simulink library "ammclib_bam_S32K3xx"  (R2016a)
(part 16 of 50)

      |   f32PropGainQ=round(kpf*2^(-s16PropGainShiftQ)*2^31);
      |   if f32PropGainQ>2^31-1
      |     f32PropGainQ=2^31-1;
      |     warning(['Parameter f32PropGainQ of ' gcb ' exceeds the fixed-point range.']);
      |   end
      |   if f32PropGainQ<-2^31
      |     f32PropGainQ=-2^31;
      |     warning(['Parameter f32PropGainQ of ' gcb ' exceeds the fixed-point range.']);
      |   end
      |   kif=igain*SampleTime*0.5*wmax/iscale;
      |   s16IntegGainShiftQ=ceil(log2(abs(kif)));
      |   if s16IntegGainShiftQ<-31
      |     s16IntegGainShiftQ=-31;
      |   end
      |   if s16IntegGainShiftQ>31
      |     s16IntegGainShiftQ=31;
      |     warning(['Parameter s16IntegGainShiftQ of ' gcb ' exceeds the fixed-point range.']);
      |   end
      |   f32IntegGainQ=round(kif*2^(-s16IntegGainShiftQ)*2^31);
      |   if f32IntegGainQ>2^31-1
      |     f32IntegGainQ=2^31-1;
      |     warning(['Parameter f32IntegGainQ of ' gcb ' exceeds the fixed-point range.']);
      |   end
      |   if f32IntegGainQ<-2^31
      |     f32IntegGainQ=-2^31;
      |     warning(['Parameter f32IntegGainQ of ' gcb ' exceeds the fixed-point range.']);
      |   end
      |   f32LowerLimitQ=-2147483648;
      |   f32UpperLimitQ=2147483647;
      |   fwkpf=0.9*pgain*wmax/iscale;
      |   s16PropGainShiftFW=ceil(log2(abs(fwkpf)));
      |   if s16PropGainShiftFW<-31
      |     s16PropGainShiftFW=-31;
      |   end
      |   if s16PropGainShiftFW>31
      |     s16PropGainShiftFW=31;
      |     warning(['Parameter s16PropGainShiftFW of ' gcb ' exceeds the fixed-point range.']);
      |   end
      |   f32PropGainFW=round(fwkpf*2^(-s16PropGainShiftFW)*2^31);
      |   if f32PropGainFW>2^31-1
      |     f32PropGainFW=2^31-1;
      |     warning(['Parameter f32PropGainFW of ' gcb ' exceeds the fixed-point range.']);
      |   end
      |   if f32PropGainFW<-2^31
      |     f32PropGainFW=-2^31;
      |     warning(['Parameter f32PropGainFW of ' gcb ' exceeds the fixed-point range.']);
      |   end
      |   s16IntegGainShiftFW=s16IntegGainShiftQ;
      |   f32IntegGainFW=f32IntegGainQ;
      |   if (Idmax<0)
      |     iratio=abs(Idmax)/iscale;
      |     if (abs(iratio) > 1)
      |       iratio = 0;
      |     end
      |     lowlim=0.3183098861837907*acos(iratio)-0.5;
      |   else
      |     lowlim=0.0;
      |   end
      |   f32LowerLimitFW=round(lowlim*2^31);
      |   if f32LowerLimitFW>2^31-1
      |     f32LowerLimitFW=2^31-1;
      |     warning(['Parameter f32LowerLimitFW of ' gcb ' exceeds the fixed-point range.']);
      |   end
      |   if f32LowerLimitFW<-2^31
      |     f32LowerLimitFW=-2^31;
      |     warning(['Parameter f32LowerLimitFW of ' gcb ' exceeds the fixed-point range.']);
      |   end
      |   f32UpperLimitFW=0;
      |   u16NSamplesW=round(log2(1.0/abs(lambdaW)));
      |   if u16NSamplesW>31
      |     u16NSamplesW=31;
      |   end
      |   if u16NSamplesW<0
      |     u16NSamplesW=0;
      |   end
      |   u16NSamplesFW=round(log2(1.0/abs(lambdaFW)));
      |   if u16NSamplesFW>31
      |     u16NSamplesFW=31;
      |   end
      |   if u16NSamplesFW<0
      |     u16NSamplesFW=0;
      |   end
      |   rampsc=polepairs*abs(ramprpm)*0.1047197551196598/wmax;
      |   f32RampUp=round(rampsc*2^31);
      |   if f32RampUp>2^31-1
      |     f32RampUp=2^31-1;
      |     warning(['Parameter f32RampUp of ' gcb ' exceeds the fixed-point range.']);
      |   end
      |   if f32RampUp<-2^31
      |     f32RampUp=-2^31;
      |     warning(['Parameter f32RampUp of ' gcb ' exceeds the fixed-point range.']);
      |   end
      |   f32RampDown=round(rampsc*2^31);
      |   if f32RampDown>2^31-1
      |     f32RampDown=2^31-1;
      |     warning(['Parameter f32RampDown of ' gcb ' exceeds the fixed-point range.']);
      |   end
      |   if f32RampDown<-2^31
      |     f32RampDown=-2^31;
      |     warning(['Parameter f32RampDown of ' gcb ' exceeds the fixed-point range.']);
      |   end
      |   if isnan(u16NSamplesW)
      |     if ~strcmp(u16NSamplesW_bkup,'0')
      |       set_param(gcb,'u16NSamplesW','0');
      |     end
      |   else
      |     tmps=num2str(u16NSamplesW);
      |     if ~strcmp(u16NSamplesW_bkup,tmps)
      |       set_param(gcb,'u16NSamplesW',tmps);
      |     end
      |   end
      |   if isnan(u16NSamplesFW)
      |     if ~strcmp(u16NSamplesFW_bkup,'0')
      |       set_param(gcb,'u16NSamplesFW','0');
      |     end
      |   else
      |     tmps=num2str(u16NSamplesFW);
      |     if ~strcmp(u16NSamplesFW_bkup,tmps)
      |       set_param(gcb,'u16NSamplesFW',tmps);
      |     end
      |   end
      |   if isnan(f32PropGainQ)
      |     if ~strcmp(f32PropGainQ_bkup,'0')
      |       set_param(gcb,'f32PropGainQ','0');
      |     end
      |   else
      |     tmps=num2str(f32PropGainQ);
      |     if ~strcmp(f32PropGainQ_bkup,tmps)
      |       set_param(gcb,'f32PropGainQ',tmps);
      |     end
      |   end
      |   if isnan(f32IntegGainQ)
      |     if ~strcmp(f32IntegGainQ_bkup,'0')
      |       set_param(gcb,'f32IntegGainQ','0');
      |     end
      |   else
      |     tmps=num2str(f32IntegGainQ);
      |     if ~strcmp(f32IntegGainQ_bkup,tmps)
      |       set_param(gcb,'f32IntegGainQ',tmps);
      |     end
      |   end
      |   if isnan(s16PropGainShiftQ)
      |     if ~strcmp(s16PropGainShiftQ_bkup,'0')
      |       set_param(gcb,'s16PropGainShiftQ','0');
      |     end
      |   else
      |     tmps=num2str(s16PropGainShiftQ);
      |     if ~strcmp(s16PropGainShiftQ_bkup,tmps)
      |       set_param(gcb,'s16PropGainShiftQ',tmps);
      |     end
      |   end
      |   if isnan(s16IntegGainShiftQ)
      |     if ~strcmp(s16IntegGainShiftQ_bkup,'0')
      |       set_param(gcb,'s16IntegGainShiftQ','0');
      |     end
      |   else
      |     tmps=num2str(s16IntegGainShiftQ);
      |     if ~strcmp(s16IntegGainShiftQ_bkup,tmps)
      |       set_param(gcb,'s16IntegGainShiftQ',tmps);
      |     end
      |   end
      |   if isnan(f32LowerLimitQ)
      |     if ~strcmp(f32LowerLimitQ_bkup,'0')
      |       set_param(gcb,'f32LowerLimitQ','0');
      |     end
      |   else
      |     tmps=num2str(f32LowerLimitQ);
      |     if ~strcmp(f32LowerLimitQ_bkup,tmps)
      |       set_param(gcb,'f32LowerLimitQ',tmps);
      |     end
      |   end
      |   if isnan(f32UpperLimitQ)
      |     if ~strcmp(f32UpperLimitQ_bkup,'0')
      |       set_param(gcb,'f32UpperLimitQ','0');
      |     end
      |   else
      |     tmps=num2str(f32UpperLimitQ);
      |     if ~strcmp(f32UpperLimitQ_bkup,tmps)
      |       set_param(gcb,'f32UpperLimitQ',tmps);
      |     end
      |   end
      |   if isnan(f32PropGainFW)
      |     if ~strcmp(f32PropGainFW_bkup,'0')
      |       set_param(gcb,'f32PropGainFW','0');
      |     end
      |   else
      |     tmps=num2str(f32PropGainFW);
      |     if ~strcmp(f32PropGainFW_bkup,tmps)
      |       set_param(gcb,'f32PropGainFW',tmps);
      |     end
      |   end
      |   if isnan(f32IntegGainFW)
      |     if ~strcmp(f32IntegGainFW_bkup,'0')
      |       set_param(gcb,'f32IntegGainFW','0');
      |     end
      |   else
      |     tmps=num2str(f32IntegGainFW);
      |     if ~strcmp(f32IntegGainFW_bkup,tmps)
      |       set_param(gcb,'f32IntegGainFW',tmps);
      |     end
      |   end
      |   if isnan(s16PropGainShiftFW)
      |     if ~strcmp(s16PropGainShiftFW_bkup,'0')
      |       set_param(gcb,'s16PropGainShiftFW','0');
      |     end
      |   else
      |     tmps=num2str(s16PropGainShiftFW);
      |     if ~strcmp(s16PropGainShiftFW_bkup,tmps)
      |       set_param(gcb,'s16PropGainShiftFW',tmps);
      |     end
      |   end
      |   if isnan(s16IntegGainShiftFW)
      |     if ~strcmp(s16IntegGainShiftFW_bkup,'0')
      |       set_param(gcb,'s16IntegGainShiftFW','0');
      |     end
      |   else
      |     tmps=num2str(s16IntegGainShiftFW);
      |     if ~strcmp(s16IntegGainShiftFW_bkup,tmps)
      |       set_param(gcb,'s16IntegGainShiftFW',tmps);
      |     end
      |   end
      |   if isnan(f32LowerLimitFW)
      |     if ~strcmp(f32LowerLimitFW_bkup,'0')
      |       set_param(gcb,'f32LowerLimitFW','0');
      |     end
      |   else
      |     tmps=num2str(f32LowerLimitFW);
      |     if ~strcmp(f32LowerLimitFW_bkup,tmps)
      |       set_param(gcb,'f32LowerLimitFW',tmps);
      |     end
      |   end
      |   if isnan(f32UpperLimitFW)
      |     if ~strcmp(f32UpperLimitFW_bkup,'0')
      |       set_param(gcb,'f32UpperLimitFW','0');
      |     end
      |   else
      |     tmps=num2str(f32UpperLimitFW);
      |     if ~strcmp(f32UpperLimitFW_bkup,tmps)
      |       set_param(gcb,'f32UpperLimitFW',tmps);
      |     end
      |   end
      |   if isnan(f32RampUp)
      |     if ~strcmp(f32RampUp_bkup,'0')
      |       set_param(gcb,'f32RampUp','0');
      |     end
      |   else
      |     tmps=num2str(f32RampUp);
      |     if ~strcmp(f32RampUp_bkup,tmps)
      |       set_param(gcb,'f32RampUp',tmps);
      |     end
      |   end
      |   if isnan(f32RampDown)
      |     if ~strcmp(f32RampDown_bkup,'0')
      |       set_param(gcb,'f32RampDown','0');
      |     end
      |   else
      |     tmps=num2str(f32RampDown);
      |     if ~strcmp(f32RampDown_bkup,tmps)
      |       set_param(gcb,'f32RampDown',tmps);
      |     end
      |   end
      | end
      mask Callback J:
      | autoCalcEn=get_param(gcb,'autoCalcEn');
      | if strcmp(autoCalcEn,'on')
      |   SampleTime=Simulink.data.evalinGlobal(bdroot,get_param(gcb,'SampleTime'));
      |   if (SampleTime==-1)
      |     SampleTime=str2double(get_param(gcb,'SampleTime_1'));
      |   end
      |   u16NSamplesW_bkup=get_param(gcb,'u16NSamplesW');
      |   u16NSamplesFW_bkup=get_param(gcb,'u16NSamplesFW');
      |   f32PropGainQ_bkup=get_param(gcb,'f32PropGainQ');
      |   f32IntegGainQ_bkup=get_param(gcb,'f32IntegGainQ');
      |   s16PropGainShiftQ_bkup=get_param(gcb,'s16PropGainShiftQ');
      |   s16IntegGainShiftQ_bkup=get_param(gcb,'s16IntegGainShiftQ');
      |   f32LowerLimitQ_bkup=get_param(gcb,'f32LowerLimitQ');
      |   f32UpperLimitQ_bkup=get_param(gcb,'f32UpperLimitQ');
      |   f32PropGainFW_bkup=get_param(gcb,'f32PropGainFW');
      |   f32IntegGainFW_bkup=get_param(gcb,'f32IntegGainFW');
      |   s16PropGainShiftFW_bkup=get_param(gcb,'s16PropGainShiftFW');
      |   s16IntegGainShiftFW_bkup=get_param(gcb,'s16IntegGainShiftFW');
      |   f32LowerLimitFW_bkup=get_param(gcb,'f32LowerLimitFW');
      |   f32UpperLimitFW_bkup=get_param(gcb,'f32UpperLimitFW');
      |   f32RampUp_bkup=get_param(gcb,'f32RampUp');
      |   f32RampDown_bkup=get_param(gcb,'f32RampDown');
      |   wf0=Simulink.data.evalinGlobal(bdroot,get_param(gcb,'wf0'));
      |   wksi=Simulink.data.evalinGlobal(bdroot,get_param(gcb,'wksi'));
      |   J=Simulink.data.evalinGlobal(bdroot,get_param(gcb,'J'));
      |   Kt=Simulink.data.evalinGlobal(bdroot,get_param(gcb,'Kt'));
      |   lambdaW=Simulink.data.evalinGlobal(bdroot,get_param(gcb,'lambdaW'));
      |   lambdaFW=Simulink.data.evalinGlobal(bdroot,get_param(gcb,'lambdaFW'));
      |   Idmax=Simulink.data.evalinGlobal(bdroot,get_param(gcb,'Idmax'));
      |   ramprpm=Simulink.data.evalinGlobal(bdroot,get_param(gcb,'ramprpm'));
      |   mechspeed=Simulink.data.evalinGlobal(bdroot,get_param(gcb,'mechspeed'));
      |   polepairs=Simulink.data.evalinGlobal(bdroot,get_param(gcb,'polepairs'));
      |   uscale=Simulink.data.evalinGlobal(bdroot,get_param(gcb,'uscale'));
      |   iscale=Simulink.data.evalinGlobal(bdroot,get_param(gcb,'iscale'));
      |   if (wf0<=0)
      |     warning('Natural frequency f0 must be positive.');
      |   end
      |   if (wksi<=0)
      |     warning('Current loop attenuation must be positive.');
      |   end
      |   if (wksi>1)
      |     warning('Current loop attenuation must not exceed 1.');
      |   end
      |   if (J<=0)
      |     warning('Moment of inertia J must be positive.');
      |   end
      |   if (Kt<=0)
      |     warning('Torque constant Kt must be positive.');
      |   end
      |   if (lambdaW<0)
      |     warning('MA filter smoothing factor must be in the range 0..1.');
      |   end
      |   if (lambdaW>1)
      |     warning('MA filter smoothing factor must be in the range 0..1.');
      |   end
      |   if (lambdaFW<0)
      |     warning('MA filter smoothing factor must be in the range 0..1.');
      |   end
      |   if (lambdaFW>1)
      |     warning('MA filter smoothing factor must be in the range 0..1.');
      |   end
      |   if (mechspeed<=0)
      |     warning('Max. speed must be positive.');
      |   end
      |   if (polepairs<1)
      |     warning('Number of pole pairs must be a natural number (1, 2, 3, ...).');
      |   end
      |   if (round(polepairs)~=polepairs)
      |     warning('Number of pole pairs must be a natural number (1, 2, 3, ...).');
      |   end
      |   if (uscale<=0)
      |     warning('U_max must be positive.');
      |   end
      |   if (iscale<=0)
      |     warning('I_max must be positive.');
      |   end
      |   w0=6.283185307179586*wf0;
      |   pgain=2.0*wksi*w0*J/Kt;
      |   igain=w0*w0*J/Kt;
      |   wmax=polepairs*mechspeed*0.1047197551196598;
      |   kpf=pgain*wmax/iscale;
      |   s16PropGainShiftQ=ceil(log2(abs(kpf)));
      |   if s16PropGainShiftQ<-31
      |     s16PropGainShiftQ=-31;
      |   end
      |   if s16PropGainShiftQ>31
      |     s16PropGainShiftQ=31;
      |     warning(['Parameter s16PropGainShiftQ of ' gcb ' exceeds the fixed-point range.']);
      |   end
      |   f32PropGainQ=round(kpf*2^(-s16PropGainShiftQ)*2^31);
      |   if f32PropGainQ>2^31-1
      |     f32PropGainQ=2^31-1;
      |     warning(['Parameter f32PropGainQ of ' gcb ' exceeds the fixed-point range.']);
      |   end
      |   if f32PropGainQ<-2^31
      |     f32PropGainQ=-2^31;
      |     warning(['Parameter f32PropGainQ of ' gcb ' exceeds the fixed-point range.']);
      |   end
      |   kif=igain*SampleTime*0.5*wmax/iscale;
      |   s16IntegGainShiftQ=ceil(log2(abs(kif)));
      |   if s16IntegGainShiftQ<-31
      |     s16IntegGainShiftQ=-31;
      |   end
      |   if s16IntegGainShiftQ>31
      |     s16IntegGainShiftQ=31;
      |     warning(['Parameter s16IntegGainShiftQ of ' gcb ' exceeds the fixed-point range.']);
      |   end
      |   f32IntegGainQ=round(kif*2^(-s16IntegGainShiftQ)*2^31);
      |   if f32IntegGainQ>2^31-1
      |     f32IntegGainQ=2^31-1;
      |     warning(['Parameter f32IntegGainQ of ' gcb ' exceeds the fixed-point range.']);
      |   end
      |   if f32IntegGainQ<-2^31
      |     f32IntegGainQ=-2^31;
      |     warning(['Parameter f32IntegGainQ of ' gcb ' exceeds the fixed-point range.']);
      |   end
      |   f32LowerLimitQ=-2147483648;
      |   f32UpperLimitQ=2147483647;
      |   fwkpf=0.9*pgain*wmax/iscale;
      |   s16PropGainShiftFW=ceil(log2(abs(fwkpf)));
      |   if s16PropGainShiftFW<-31
      |     s16PropGainShiftFW=-31;
      |   end
      |   if s16PropGainShiftFW>31
      |     s16PropGainShiftFW=31;
      |     warning(['Parameter s16PropGainShiftFW of ' gcb ' exceeds the fixed-point range.']);
      |   end
      |   f32PropGainFW=round(fwkpf*2^(-s16PropGainShiftFW)*2^31);
      |   if f32PropGainFW>2^31-1
      |     f32PropGainFW=2^31-1;
      |     warning(['Parameter f32PropGainFW of ' gcb ' exceeds the fixed-point range.']);
      |   end
      |   if f32PropGainFW<-2^31
      |     f32PropGainFW=-2^31;
      |     warning(['Parameter f32PropGainFW of ' gcb ' exceeds the fixed-point range.']);
      |   end
      |   s16IntegGainShiftFW=s16IntegGainShiftQ;
      |   f32IntegGainFW=f32IntegGainQ;
      |   if (Idmax<0)
      |     iratio=abs(Idmax)/iscale;
      |     if (abs(iratio) > 1)
      |       iratio = 0;
      |     end
      |     lowlim=0.3183098861837907*acos(iratio)-0.5;
      |   else
      |     lowlim=0.0;
      |   end
      |   f32LowerLimitFW=round(lowlim*2^31);
      |   if f32LowerLimitFW>2^31-1
      |     f32LowerLimitFW=2^31-1;
      |     warning(['Parameter f32LowerLimitFW of ' gcb ' exceeds the fixed-point range.']);
      |   end
      |   if f32LowerLimitFW<-2^31
      |     f32LowerLimitFW=-2^31;
      |     warning(['Parameter f32LowerLimitFW of ' gcb ' exceeds the fixed-point range.']);
      |   end
      |   f32UpperLimitFW=0;
      |   u16NSamplesW=round(log2(1.0/abs(lambdaW)));
      |   if u16NSamplesW>31
      |     u16NSamplesW=31;
      |   end
      |   if u16NSamplesW<0
      |     u16NSamplesW=0;
      |   end
      |   u16NSamplesFW=round(log2(1.0/abs(lambdaFW)));
      |   if u16NSamplesFW>31
      |     u16NSamplesFW=31;
      |   end
      |   if u16NSamplesFW<0
      |     u16NSamplesFW=0;
      |   end
      |   rampsc=polepairs*abs(ramprpm)*0.1047197551196598/wmax;
      |   f32RampUp=round(rampsc*2^31);
      |   if f32RampUp>2^31-1
      |     f32RampUp=2^31-1;
      |     warning(['Parameter f32RampUp of ' gcb ' exceeds the fixed-point range.']);
      |   end
      |   if f32RampUp<-2^31
      |     f32RampUp=-2^31;
      |     warning(['Parameter f32RampUp of ' gcb ' exceeds the fixed-point range.']);
      |   end
      |   f32RampDown=round(rampsc*2^31);
      |   if f32RampDown>2^31-1
      |     f32RampDown=2^31-1;
      |     warning(['Parameter f32RampDown of ' gcb ' exceeds the fixed-point range.']);
      |   end
      |   if f32RampDown<-2^31
      |     f32RampDown=-2^31;
      |     warning(['Parameter f32RampDown of ' gcb ' exceeds the fixed-point range.']);
      |   end
      |   if isnan(u16NSamplesW)
      |     if ~strcmp(u16NSamplesW_bkup,'0')
      |       set_param(gcb,'u16NSamplesW','0');
      |     end
      |   else
      |     tmps=num2str(u16NSamplesW);
      |     if ~strcmp(u16NSamplesW_bkup,tmps)
      |       set_param(gcb,'u16NSamplesW',tmps);
      |     end
      |   end
      |   if isnan(u16NSamplesFW)
      |     if ~strcmp(u16NSamplesFW_bkup,'0')
      |       set_param(gcb,'u16NSamplesFW','0');
      |     end
      |   else
      |     tmps=num2str(u16NSamplesFW);
      |     if ~strcmp(u16NSamplesFW_bkup,tmps)
      |       set_param(gcb,'u16NSamplesFW',tmps);
      |     end
      |   end
      |   if isnan(f32PropGainQ)
      |     if ~strcmp(f32PropGainQ_bkup,'0')
      |       set_param(gcb,'f32PropGainQ','0');
      |     end
      |   else
      |     tmps=num2str(f32PropGainQ);
      |     if ~strcmp(f32PropGainQ_bkup,tmps)
      |       set_param(gcb,'f32PropGainQ',tmps);
      |     end
      |   end
      |   if isnan(f32IntegGainQ)
      |     if ~strcmp(f32IntegGainQ_bkup,'0')
      |       set_param(gcb,'f32IntegGainQ','0');
      |     end
      |   else
      |     tmps=num2str(f32IntegGainQ);
      |     if ~strcmp(f32IntegGainQ_bkup,tmps)
      |       set_param(gcb,'f32IntegGainQ',tmps);
      |     end
      |   end
      |   if isnan(s16PropGainShiftQ)
      |     if ~strcmp(s16PropGainShiftQ_bkup,'0')
      |       set_param(gcb,'s16PropGainShiftQ','0');
      |     end
      |   else
      |     tmps=num2str(s16PropGainShiftQ);
      |     if ~strcmp(s16PropGainShiftQ_bkup,tmps)
      |       set_param(gcb,'s16PropGainShiftQ',tmps);
      |     end
      |   end
      |   if isnan(s16IntegGainShiftQ)
      |     if ~strcmp(s16IntegGainShiftQ_bkup,'0')
      |       set_param(gcb,'s16IntegGainShiftQ','0');
      |     end
      |   else
      |     tmps=num2str(s16IntegGainShiftQ);
      |     if ~strcmp(s16IntegGainShiftQ_bkup,tmps)
      |       set_param(gcb,'s16IntegGainShiftQ',tmps);
      |     end
      |   end
      |   if isnan(f32LowerLimitQ)
      |     if ~strcmp(f32LowerLimitQ_bkup,'0')
      |       set_param(gcb,'f32LowerLimitQ','0');
      |     end
      |   else
      |     tmps=num2str(f32LowerLimitQ);
      |     if ~strcmp(f32LowerLimitQ_bkup,tmps)
      |       set_param(gcb,'f32LowerLimitQ',tmps);
      |     end
      |   end
      |   if isnan(f32UpperLimitQ)
      |     if ~strcmp(f32UpperLimitQ_bkup,'0')
      |       set_param(gcb,'f32UpperLimitQ','0');
      |     end
      |   else
      |     tmps=num2str(f32UpperLimitQ);
      |     if ~strcmp(f32UpperLimitQ_bkup,tmps)
      |       set_param(gcb,'f32UpperLimitQ',tmps);
      |     end
      |   end
      |   if isnan(f32PropGainFW)
      |     if ~strcmp(f32PropGainFW_bkup,'0')
      |       set_param(gcb,'f32PropGainFW','0');
      |     end
      |   else
      |     tmps=num2str(f32PropGainFW);
      |     if ~strcmp(f32PropGainFW_bkup,tmps)
      |       set_param(gcb,'f32PropGainFW',tmps);
      |     end
      |   end
      |   if isnan(f32IntegGainFW)
      |     if ~strcmp(f32IntegGainFW_bkup,'0')
      |       set_param(gcb,'f32IntegGainFW','0');
      |     end
      |   else
      |     tmps=num2str(f32IntegGainFW);
      |     if ~strcmp(f32IntegGainFW_bkup,tmps)
      |       set_param(gcb,'f32IntegGainFW',tmps);
      |     end
      |   end
      |   if isnan(s16PropGainShiftFW)
      |     if ~strcmp(s16PropGainShiftFW_bkup,'0')
      |       set_param(gcb,'s16PropGainShiftFW','0');
      |     end
      |   else
      |     tmps=num2str(s16PropGainShiftFW);
      |     if ~strcmp(s16PropGainShiftFW_bkup,tmps)
      |       set_param(gcb,'s16PropGainShiftFW',tmps);
      |     end
      |   end
      |   if isnan(s16IntegGainShiftFW)
      |     if ~strcmp(s16IntegGainShiftFW_bkup,'0')
      |       set_param(gcb,'s16IntegGainShiftFW','0');
      |     end
      |   else
      |     tmps=num2str(s16IntegGainShiftFW);
      |     if ~strcmp(s16IntegGainShiftFW_bkup,tmps)
      |       set_param(gcb,'s16IntegGainShiftFW',tmps);
      |     end
      |   end
      |   if isnan(f32LowerLimitFW)
      |     if ~strcmp(f32LowerLimitFW_bkup,'0')
      |       set_param(gcb,'f32LowerLimitFW','0');
      |     end
      |   else
      |     tmps=num2str(f32LowerLimitFW);
      |     if ~strcmp(f32LowerLimitFW_bkup,tmps)
      |       set_param(gcb,'f32LowerLimitFW',tmps);
      |     end
      |   end
      |   if isnan(f32UpperLimitFW)
      |     if ~strcmp(f32UpperLimitFW_bkup,'0')
      |       set_param(gcb,'f32UpperLimitFW','0');
      |     end
      |   else
      |     tmps=num2str(f32UpperLimitFW);
      |     if ~strcmp(f32UpperLimitFW_bkup,tmps)
      |       set_param(gcb,'f32UpperLimitFW',tmps);
      |     end
      |   end
      |   if isnan(f32RampUp)
      |     if ~strcmp(f32RampUp_bkup,'0')
      |       set_param(gcb,'f32RampUp','0');
      |     end
      |   else
      |     tmps=num2str(f32RampUp);
      |     if ~strcmp(f32RampUp_bkup,tmps)
      |       set_param(gcb,'f32RampUp',tmps);
      |     end
      |   end
      |   if isnan(f32RampDown)
      |     if ~strcmp(f32RampDown_bkup,'0')
      |       set_param(gcb,'f32RampDown','0');
      |     end
      |   else
      |     tmps=num2str(f32RampDown);
      |     if ~strcmp(f32RampDown_bkup,tmps)
      |       set_param(gcb,'f32RampDown',tmps);
      |     end
      |   end
      | end
      mask Callback Kt:
      | autoCalcEn=get_param(gcb,'autoCalcEn');
      | if strcmp(autoCalcEn,'on')
      |   SampleTime=Simulink.data.evalinGlobal(bdroot,get_param(gcb,'SampleTime'));
      |   if (SampleTime==-1)
      |     SampleTime=str2double(get_param(gcb,'SampleTime_1'));
      |   end
      |   u16NSamplesW_bkup=get_param(gcb,'u16NSamplesW');
      |   u16NSamplesFW_bkup=get_param(gcb,'u16NSamplesFW');
      |   f32PropGainQ_bkup=get_param(gcb,'f32PropGainQ');
      |   f32IntegGainQ_bkup=get_param(gcb,'f32IntegGainQ');
      |   s16PropGainShiftQ_bkup=get_param(gcb,'s16PropGainShiftQ');
      |   s16IntegGainShiftQ_bkup=get_param(gcb,'s16IntegGainShiftQ');
      |   f32LowerLimitQ_bkup=get_param(gcb,'f32LowerLimitQ');
      |   f32UpperLimitQ_bkup=get_param(gcb,'f32UpperLimitQ');
      |   f32PropGainFW_bkup=get_param(gcb,'f32PropGainFW');
      |   f32IntegGainFW_bkup=get_param(gcb,'f32IntegGainFW');
      |   s16PropGainShiftFW_bkup=get_param(gcb,'s16PropGainShiftFW');
      |   s16IntegGainShiftFW_bkup=get_param(gcb,'s16IntegGainShiftFW');
      |   f32LowerLimitFW_bkup=get_param(gcb,'f32LowerLimitFW');
      |   f32UpperLimitFW_bkup=get_param(gcb,'f32UpperLimitFW');
      |   f32RampUp_bkup=get_param(gcb,'f32RampUp');
      |   f32RampDown_bkup=get_param(gcb,'f32RampDown');
      |   wf0=Simulink.data.evalinGlobal(bdroot,get_param(gcb,'wf0'));
      |   wksi=Simulink.data.evalinGlobal(bdroot,get_param(gcb,'wksi'));
      |   J=Simulink.data.evalinGlobal(bdroot,get_param(gcb,'J'));
      |   Kt=Simulink.data.evalinGlobal(bdroot,get_param(gcb,'Kt'));
      |   lambdaW=Simulink.data.evalinGlobal(bdroot,get_param(gcb,'lambdaW'));
      |   lambdaFW=Simulink.data.evalinGlobal(bdroot,get_param(gcb,'lambdaFW'));
      |   Idmax=Simulink.data.evalinGlobal(bdroot,get_param(gcb,'Idmax'));
      |   ramprpm=Simulink.data.evalinGlobal(bdroot,get_param(gcb,'ramprpm'));
      |   mechspeed=Simulink.data.evalinGlobal(bdroot,get_param(gcb,'mechspeed'));
      |   polepairs=Simulink.data.evalinGlobal(bdroot,get_param(gcb,'polepairs'));
      |   uscale=Simulink.data.evalinGlobal(bdroot,get_param(gcb,'uscale'));
      |   iscale=Simulink.data.evalinGlobal(bdroot,get_param(gcb,'iscale'));
      |   if (wf0<=0)
      |     warning('Natural frequency f0 must be positive.');
      |   end
      |   if (wksi<=0)
      |     warning('Current loop attenuation must be positive.');
      |   end
      |   if (wksi>1)
      |     warning('Current loop attenuation must not exceed 1.');
      |   end
      |   if (J<=0)
      |     warning('Moment of inertia J must be positive.');
      |   end
      |   if (Kt<=0)
      |     warning('Torque constant Kt must be positive.');
      |   end
      |   if (lambdaW<0)
      |     warning('MA filter smoothing factor must be in the range 0..1.');
      |   end
      |   if (lambdaW>1)
      |     warning('MA filter smoothing factor must be in the range 0..1.');
      |   end
      |   if (lambdaFW<0)
      |     warning('MA filter smoothing factor must be in the range 0..1.');
      |   end
      |   if (lambdaFW>1)
      |     warning('MA filter smoothing factor must be in the range 0..1.');
      |   end
      |   if (mechspeed<=0)
      |     warning('Max. speed must be positive.');
      |   end
      |   if (polepairs<1)
      |     warning('Number of pole pairs must be a natural number (1, 2, 3, ...).');
      |   end
      |   if (round(polepairs)~=polepairs)
      |     warning('Number of pole pairs must be a natural number (1, 2, 3, ...).');
      |   end
      |   if (uscale<=0)
      |     warning('U_max must be positive.');
      |   end
      |   if (iscale<=0)
      |     warning('I_max must be positive.');
      |   end
      |   w0=6.283185307179586*wf0;
      |   pgain=2.0*wksi*w0*J/Kt;
      |   igain=w0*w0*J/Kt;
      |   wmax=polepairs*mechspeed*0.1047197551196598;
      |   kpf=pgain*wmax/iscale;
      |   s16PropGainShiftQ=ceil(log2(abs(kpf)));
      |   if s16PropGainShiftQ<-31
      |     s16PropGainShiftQ=-31;
      |   end
      |   if s16PropGainShiftQ>31
      |     s16PropGainShiftQ=31;
      |     warning(['Parameter s16PropGainShiftQ of ' gcb ' exceeds the fixed-point range.']);
      |   end
      |   f32PropGainQ=round(kpf*2^(-s16PropGainShiftQ)*2^31);
      |   if f32PropGainQ>2^31-1
      |     f32PropGainQ=2^31-1;
      |     warning(['Parameter f32PropGainQ of ' gcb ' exceeds the fixed-point range.']);
      |   end
      |   if f32PropGainQ<-2^31
      |     f32PropGainQ=-2^31;
      |     warning(['Parameter f32PropGainQ of ' gcb ' exceeds the fixed-point range.']);
      |   end
      |   kif=igain*SampleTime*0.5*wmax/iscale;
      |   s16IntegGainShiftQ=ceil(log2(abs(kif)));
      |   if s16IntegGainShiftQ<-31
      |     s16IntegGainShiftQ=-31;
      |   end
      |   if s16IntegGainShiftQ>31
      |     s16IntegGainShiftQ=31;
      |     warning(['Parameter s16IntegGainShiftQ of ' gcb ' exceeds the fixed-point range.']);
      |   end
      |   f32IntegGainQ=round(kif*2^(-s16IntegGainShiftQ)*2^31);
      |   if f32IntegGainQ>2^31-1
      |     f32IntegGainQ=2^31-1;
      |     warning(['Parameter f32IntegGainQ of ' gcb ' exceeds the fixed-point range.']);
      |   end
      |   if f32IntegGainQ<-2^31
      |     f32IntegGainQ=-2^31;
      |     warning(['Parameter f32IntegGainQ of ' gcb ' exceeds the fixed-point range.']);
      |   end
      |   f32LowerLimitQ=-2147483648;
      |   f32UpperLimitQ=2147483647;
      |   fwkpf=0.9*pgain*wmax/iscale;
      |   s16PropGainShiftFW=ceil(log2(abs(fwkpf)));
      |   if s16PropGainShiftFW<-31
      |     s16PropGainShiftFW=-31;
      |   end
      |   if s16PropGainShiftFW>31
      |     s16PropGainShiftFW=31;
      |     warning(['Parameter s16PropGainShiftFW of ' gcb ' exceeds the fixed-point range.']);
      |   end
      |   f32PropGainFW=round(fwkpf*2^(-s16PropGainShiftFW)*2^31);
      |   if f32PropGainFW>2^31-1
      |     f32PropGainFW=2^31-1;
      |     warning(['Parameter f32PropGainFW of ' gcb ' exceeds the fixed-point range.']);
      |   end
      |   if f32PropGainFW<-2^31
      |     f32PropGainFW=-2^31;
      |     warning(['Parameter f32PropGainFW of ' gcb ' exceeds the fixed-point range.']);
      |   end
      |   s16IntegGainShiftFW=s16IntegGainShiftQ;
      |   f32IntegGainFW=f32IntegGainQ;
      |   if (Idmax<0)
      |     iratio=abs(Idmax)/iscale;
      |     if (abs(iratio) > 1)
      |       iratio = 0;
      |     end
      |     lowlim=0.3183098861837907*acos(iratio)-0.5;
      |   else
      |     lowlim=0.0;
      |   end
      |   f32LowerLimitFW=round(lowlim*2^31);
      |   if f32LowerLimitFW>2^31-1
      |     f32LowerLimitFW=2^31-1;
      |     warning(['Parameter f32LowerLimitFW of ' gcb ' exceeds the fixed-point range.']);
      |   end
      |   if f32LowerLimitFW<-2^31
      |     f32LowerLimitFW=-2^31;
      |     warning(['Parameter f32LowerLimitFW of ' gcb ' exceeds the fixed-point range.']);
      |   end
      |   f32UpperLimitFW=0;
      |   u16NSamplesW=round(log2(1.0/abs(lambdaW)));
      |   if u16NSamplesW>31
      |     u16NSamplesW=31;
      |   end
      |   if u16NSamplesW<0
      |     u16NSamplesW=0;
      |   end
      |   u16NSamplesFW=round(log2(1.0/abs(lambdaFW)));
      |   if u16NSamplesFW>31
      |     u16NSamplesFW=31;
      |   end
      |   if u16NSamplesFW<0
      |     u16NSamplesFW=0;
      |   end
      |   rampsc=polepairs*abs(ramprpm)*0.1047197551196598/wmax;
      |   f32RampUp=round(rampsc*2^31);
      |   if f32RampUp>2^31-1
      |     f32RampUp=2^31-1;
      |     warning(['Parameter f32RampUp of ' gcb ' exceeds the fixed-point range.']);
      |   end
      |   if f32RampUp<-2^31
      |     f32RampUp=-2^31;
      |     warning(['Parameter f32RampUp of ' gcb ' exceeds the fixed-point range.']);
      |   end
      |   f32RampDown=round(rampsc*2^31);
      |   if f32RampDown>2^31-1
      |     f32RampDown=2^31-1;
      |     warning(['Parameter f32RampDown of ' gcb ' exceeds the fixed-point range.']);
      |   end
      |   if f32RampDown<-2^31
      |     f32RampDown=-2^31;
      |     warning(['Parameter f32RampDown of ' gcb ' exceeds the fixed-point range.']);
      |   end
      |   if isnan(u16NSamplesW)
      |     if ~strcmp(u16NSamplesW_bkup,'0')
      |       set_param(gcb,'u16NSamplesW','0');
      |     end
      |   else
      |     tmps=num2str(u16NSamplesW);
      |     if ~strcmp(u16NSamplesW_bkup,tmps)
      |       set_param(gcb,'u16NSamplesW',tmps);
      |     end
      |   end
      |   if isnan(u16NSamplesFW)
      |     if ~strcmp(u16NSamplesFW_bkup,'0')
      |       set_param(gcb,'u16NSamplesFW','0');
      |     end
      |   else
      |     tmps=num2str(u16NSamplesFW);
      |     if ~strcmp(u16NSamplesFW_bkup,tmps)
      |       set_param(gcb,'u16NSamplesFW',tmps);
      |     end
      |   end
      |   if isnan(f32PropGainQ)
      |     if ~strcmp(f32PropGainQ_bkup,'0')
      |       set_param(gcb,'f32PropGainQ','0');
      |     end
      |   else
      |     tmps=num2str(f32PropGainQ);
      |     if ~strcmp(f32PropGainQ_bkup,tmps)
      |       set_param(gcb,'f32PropGainQ',tmps);
      |     end
      |   end
      |   if isnan(f32IntegGainQ)
      |     if ~strcmp(f32IntegGainQ_bkup,'0')
      |       set_param(gcb,'f32IntegGainQ','0');
      |     end
      |   else
      |     tmps=num2str(f32IntegGainQ);
      |     if ~strcmp(f32IntegGainQ_bkup,tmps)
      |       set_param(gcb,'f32IntegGainQ',tmps);
      |     end
      |   end
      |   if isnan(s16PropGainShiftQ)
      |     if ~strcmp(s16PropGainShiftQ_bkup,'0')
      |       set_param(gcb,'s16PropGainShiftQ','0');
      |     end
      |   else
      |     tmps=num2str(s16PropGainShiftQ);
      |     if ~strcmp(s16PropGainShiftQ_bkup,tmps)
      |       set_param(gcb,'s16PropGainShiftQ',tmps);
      |     end
      |   end
      |   if isnan(s16IntegGainShiftQ)
      |     if ~strcmp(s16IntegGainShiftQ_bkup,'0')
      |       set_param(gcb,'s16IntegGainShiftQ','0');
      |     end
      |   else
      |     tmps=num2str(s16IntegGainShiftQ);
      |     if ~strcmp(s16IntegGainShiftQ_bkup,tmps)
      |       set_param(gcb,'s16IntegGainShiftQ',tmps);
      |     end
      |   end
      |   if isnan(f32LowerLimitQ)
      |     if ~strcmp(f32LowerLimitQ_bkup,'0')
      |       set_param(gcb,'f32LowerLimitQ','0');
      |     end
      |   else
      |     tmps=num2str(f32LowerLimitQ);
      |     if ~strcmp(f32LowerLimitQ_bkup,tmps)
      |       set_param(gcb,'f32LowerLimitQ',tmps);
      |     end
      |   end
      |   if isnan(f32UpperLimitQ)
      |     if ~strcmp(f32UpperLimitQ_bkup,'0')
      |       set_param(gcb,'f32UpperLimitQ','0');
      |     end
      |   else
      |     tmps=num2str(f32UpperLimitQ);
      |     if ~strcmp(f32UpperLimitQ_bkup,tmps)
      |       set_param(gcb,'f32UpperLimitQ',tmps);
      |     end
      |   end
      |   if isnan(f32PropGainFW)
      |     if ~strcmp(f32PropGainFW_bkup,'0')
      |       set_param(gcb,'f32PropGainFW','0');
      |     end
      |   else
      |     tmps=num2str(f32PropGainFW);
      |     if ~strcmp(f32PropGainFW_bkup,tmps)
      |       set_param(gcb,'f32PropGainFW',tmps);
      |     end
      |   end
      |   if isnan(f32IntegGainFW)
      |     if ~strcmp(f32IntegGainFW_bkup,'0')
      |       set_param(gcb,'f32IntegGainFW','0');
      |     end
      |   else
      |     tmps=num2str(f32IntegGainFW);
      |     if ~strcmp(f32IntegGainFW_bkup,tmps)
      |       set_param(gcb,'f32IntegGainFW',tmps);
      |     end
      |   end
      |   if isnan(s16PropGainShiftFW)
      |     if ~strcmp(s16PropGainShiftFW_bkup,'0')
      |       set_param(gcb,'s16PropGainShiftFW','0');
      |     end
      |   else
      |     tmps=num2str(s16PropGainShiftFW);
      |     if ~strcmp(s16PropGainShiftFW_bkup,tmps)
      |       set_param(gcb,'s16PropGainShiftFW',tmps);
      |     end
      |   end
      |   if isnan(s16IntegGainShiftFW)
      |     if ~strcmp(s16IntegGainShiftFW_bkup,'0')
      |       set_param(gcb,'s16IntegGainShiftFW','0');
      |     end
      |   else
      |     tmps=num2str(s16IntegGainShiftFW);
      |     if ~strcmp(s16IntegGainShiftFW_bkup,tmps)
      |       set_param(gcb,'s16IntegGainShiftFW',tmps);
      |     end
      |   end
      |   if isnan(f32LowerLimitFW)
      |     if ~strcmp(f32LowerLimitFW_bkup,'0')
      |       set_param(gcb,'f32LowerLimitFW','0');
      |     end
      |   else
      |     tmps=num2str(f32LowerLimitFW);
      |     if ~strcmp(f32LowerLimitFW_bkup,tmps)
      |       set_param(gcb,'f32LowerLimitFW',tmps);
      |     end
      |   end
      |   if isnan(f32UpperLimitFW)
      |     if ~strcmp(f32UpperLimitFW_bkup,'0')
      |       set_param(gcb,'f32UpperLimitFW','0');
      |     end
      |   else
      |     tmps=num2str(f32UpperLimitFW);
      |     if ~strcmp(f32UpperLimitFW_bkup,tmps)
      |       set_param(gcb,'f32UpperLimitFW',tmps);
      |     end
      |   end
      |   if isnan(f32RampUp)
      |     if ~strcmp(f32RampUp_bkup,'0')
      |       set_param(gcb,'f32RampUp','0');
      |     end
      |   else
      |     tmps=num2str(f32RampUp);
      |     if ~strcmp(f32RampUp_bkup,tmps)
      |       set_param(gcb,'f32RampUp',tmps);
      |     end
      |   end
      |   if isnan(f32RampDown)
      |     if ~strcmp(f32RampDown_bkup,'0')
      |       set_param(gcb,'f32RampDown','0');
      |     end
      |   else
      |     tmps=num2str(f32RampDown);
      |     if ~strcmp(f32RampDown_bkup,tmps)
      |       set_param(gcb,'f32RampDown',tmps);
      |     end
      |   end
      | end
      mask Callback lambdaW:
      | autoCalcEn=get_param(gcb,'autoCalcEn');
      | if strcmp(autoCalcEn,'on')
      |   SampleTime=Simulink.data.evalinGlobal(bdroot,get_param(gcb,'SampleTime'));
      |   if (SampleTime==-1)
      |     SampleTime=str2double(get_param(gcb,'SampleTime_1'));
      |   end
      |   u16NSamplesW_bkup=get_param(gcb,'u16NSamplesW');
      |   u16NSamplesFW_bkup=get_param(gcb,'u16NSamplesFW');
      |   f32PropGainQ_bkup=get_param(gcb,'f32PropGainQ');
      |   f32IntegGainQ_bkup=get_param(gcb,'f32IntegGainQ');
      |   s16PropGainShiftQ_bkup=get_param(gcb,'s16PropGainShiftQ');
      |   s16IntegGainShiftQ_bkup=get_param(gcb,'s16IntegGainShiftQ');
      |   f32LowerLimitQ_bkup=get_param(gcb,'f32LowerLimitQ');
      |   f32UpperLimitQ_bkup=get_param(gcb,'f32UpperLimitQ');
      |   f32PropGainFW_bkup=get_param(gcb,'f32PropGainFW');
      |   f32IntegGainFW_bkup=get_param(gcb,'f32IntegGainFW');
      |   s16PropGainShiftFW_bkup=get_param(gcb,'s16PropGainShiftFW');
      |   s16IntegGainShiftFW_bkup=get_param(gcb,'s16IntegGainShiftFW');
      |   f32LowerLimitFW_bkup=get_param(gcb,'f32LowerLimitFW');
      |   f32UpperLimitFW_bkup=get_param(gcb,'f32UpperLimitFW');
      |   f32RampUp_bkup=get_param(gcb,'f32RampUp');
      |   f32RampDown_bkup=get_param(gcb,'f32RampDown');
      |   wf0=Simulink.data.evalinGlobal(bdroot,get_param(gcb,'wf0'));
      |   wksi=Simulink.data.evalinGlobal(bdroot,get_param(gcb,'wksi'));
      |   J=Simulink.data.evalinGlobal(bdroot,get_param(gcb,'J'));
      |   Kt=Simulink.data.evalinGlobal(bdroot,get_param(gcb,'Kt'));
      |   lambdaW=Simulink.data.evalinGlobal(bdroot,get_param(gcb,'lambdaW'));
      |   lambdaFW=Simulink.data.evalinGlobal(bdroot,get_param(gcb,'lambdaFW'));
      |   Idmax=Simulink.data.evalinGlobal(bdroot,get_param(gcb,'Idmax'));
      |   ramprpm=Simulink.data.evalinGlobal(bdroot,get_param(gcb,'ramprpm'));
      |   mechspeed=Simulink.data.evalinGlobal(bdroot,get_param(gcb,'mechspeed'));
      |   polepairs=Simulink.data.evalinGlobal(bdroot,get_param(gcb,'polepairs'));
      |   uscale=Simulink.data.evalinGlobal(bdroot,get_param(gcb,'uscale'));
      |   iscale=Simulink.data.evalinGlobal(bdroot,get_param(gcb,'iscale'));
      |   if (wf0<=0)
      |     warning('Natural frequency f0 must be positive.');
      |   end
      |   if (wksi<=0)
      |     warning('Current loop attenuation must be positive.');
      |   end
      |   if (wksi>1)
      |     warning('Current loop attenuation must not exceed 1.');
      |   end
      |   if (J<=0)
      |     warning('Moment of inertia J must be positive.');
      |   end
      |   if (Kt<=0)
      |     warning('Torque constant Kt must be positive.');
      |   end
      |   if (lambdaW<0)
      |     warning('MA filter smoothing factor must be in the range 0..1.');
      |   end
      |   if (lambdaW>1)
      |     warning('MA filter smoothing factor must be in the range 0..1.');
      |   end
      |   if (lambdaFW<0)
      |     warning('MA filter smoothing factor must be in the range 0..1.');
      |   end
      |   if (lambdaFW>1)
      |     warning('MA filter smoothing factor must be in the range 0..1.');
      |   end
      |   if (mechspeed<=0)
      |     warning('Max. speed must be positive.');
      |   end
      |   if (polepairs<1)
      |     warning('Number of pole pairs must be a natural number (1, 2, 3, ...).');
      |   end
      |   if (round(polepairs)~=polepairs)
      |     warning('Number of pole pairs must be a natural number (1, 2, 3, ...).');
      |   end
      |   if (uscale<=0)
      |     warning('U_max must be positive.');
      |   end
      |   if (iscale<=0)
      |     warning('I_max must be positive.');
      |   end
      |   w0=6.283185307179586*wf0;
      |   pgain=2.0*wksi*w0*J/Kt;
      |   igain=w0*w0*J/Kt;
      |   wmax=polepairs*mechspeed*0.1047197551196598;
      |   kpf=pgain*wmax/iscale;
      |   s16PropGainShiftQ=ceil(log2(abs(kpf)));
      |   if s16PropGainShiftQ<-31
      |     s16PropGainShiftQ=-31;
      |   end
      |   if s16PropGainShiftQ>31
      |     s16PropGainShiftQ=31;
      |     warning(['Parameter s16PropGainShiftQ of ' gcb ' exceeds the fixed-point range.']);
      |   end
      |   f32PropGainQ=round(kpf*2^(-s16PropGainShiftQ)*2^31);
      |   if f32PropGainQ>2^31-1
      |     f32PropGainQ=2^31-1;
      |     warning(['Parameter f32PropGainQ of ' gcb ' exceeds the fixed-point range.']);
      |   end
      |   if f32PropGainQ<-2^31
      |     f32PropGainQ=-2^31;
      |     warning(['Parameter f32PropGainQ of ' gcb ' exceeds the fixed-point range.']);
      |   end
      |   kif=igain*SampleTime*0.5*wmax/iscale;
      |   s16IntegGainShiftQ=ceil(log2(abs(kif)));
      |   if s16IntegGainShiftQ<-31
      |     s16IntegGainShiftQ=-31;
      |   end
      |   if s16IntegGainShiftQ>31
      |     s16IntegGainShiftQ=31;
      |     warning(['Parameter s16IntegGainShiftQ of ' gcb ' exceeds the fixed-point range.']);
      |   end
      |   f32IntegGainQ=round(kif*2^(-s16IntegGainShiftQ)*2^31);
      |   if f32IntegGainQ>2^31-1
      |     f32IntegGainQ=2^31-1;
      |     warning(['Parameter f32IntegGainQ of ' gcb ' exceeds the fixed-point range.']);
      |   end
      |   if f32IntegGainQ<-2^31
      |     f32IntegGainQ=-2^31;
      |     warning(['Parameter f32IntegGainQ of ' gcb ' exceeds the fixed-point range.']);
      |   end
      |   f32LowerLimitQ=-2147483648;
      |   f32UpperLimitQ=2147483647;
      |   fwkpf=0.9*pgain*wmax/iscale;
      |   s16PropGainShiftFW=ceil(log2(abs(fwkpf)));
      |   if s16PropGainShiftFW<-31
      |     s16PropGainShiftFW=-31;
      |   end
      |   if s16PropGainShiftFW>31
      |     s16PropGainShiftFW=31;
      |     warning(['Parameter s16PropGainShiftFW of ' gcb ' exceeds the fixed-point range.']);
      |   end
      |   f32PropGainFW=round(fwkpf*2^(-s16PropGainShiftFW)*2^31);
      |   if f32PropGainFW>2^31-1
      |     f32PropGainFW=2^31-1;
      |     warning(['Parameter f32PropGainFW of ' gcb ' exceeds the fixed-point range.']);
      |   end
      |   if f32PropGainFW<-2^31
      |     f32PropGainFW=-2^31;
      |     warning(['Parameter f32PropGainFW of ' gcb ' exceeds the fixed-point range.']);
      |   end
      |   s16IntegGainShiftFW=s16IntegGainShiftQ;
      |   f32IntegGainFW=f32IntegGainQ;
      |   if (Idmax<0)
      |     iratio=abs(Idmax)/iscale;
      |     if (abs(iratio) > 1)
      |       iratio = 0;
      |     end
      |     lowlim=0.3183098861837907*acos(iratio)-0.5;
      |   else
      |     lowlim=0.0;
      |   end
      |   f32LowerLimitFW=round(lowlim*2^31);
      |   if f32LowerLimitFW>2^31-1
      |     f32LowerLimitFW=2^31-1;
      |     warning(['Parameter f32LowerLimitFW of ' gcb ' exceeds the fixed-point range.']);
      |   end
      |   if f32LowerLimitFW<-2^31
      |     f32LowerLimitFW=-2^31;
      |     warning(['Parameter f32LowerLimitFW of ' gcb ' exceeds the fixed-point range.']);
      |   end
      |   f32UpperLimitFW=0;
      |   u16NSamplesW=round(log2(1.0/abs(lambdaW)));
      |   if u16NSamplesW>31
      |     u16NSamplesW=31;
      |   end
      |   if u16NSamplesW<0
      |     u16NSamplesW=0;
      |   end
      |   u16NSamplesFW=round(log2(1.0/abs(lambdaFW)));
      |   if u16NSamplesFW>31
      |     u16NSamplesFW=31;
      |   end
      |   if u16NSamplesFW<0
      |     u16NSamplesFW=0;
      |   end
      |   rampsc=polepairs*abs(ramprpm)*0.1047197551196598/wmax;
      |   f32RampUp=round(rampsc*2^31);
      |   if f32RampUp>2^31-1
      |     f32RampUp=2^31-1;
      |     warning(['Parameter f32RampUp of ' gcb ' exceeds the fixed-point range.']);
      |   end
      |   if f32RampUp<-2^31
      |     f32RampUp=-2^31;
      |     warning(['Parameter f32RampUp of ' gcb ' exceeds the fixed-point range.']);
      |   end
      |   f32RampDown=round(rampsc*2^31);
      |   if f32RampDown>2^31-1
      |     f32RampDown=2^31-1;
      |     warning(['Parameter f32RampDown of ' gcb ' exceeds the fixed-point range.']);
      |   end
      |   if f32RampDown<-2^31
      |     f32RampDown=-2^31;
      |     warning(['Parameter f32RampDown of ' gcb ' exceeds the fixed-point range.']);
      |   end
      |   if isnan(u16NSamplesW)
      |     if ~strcmp(u16NSamplesW_bkup,'0')
      |       set_param(gcb,'u16NSamplesW','0');
      |     end
      |   else
      |     tmps=num2str(u16NSamplesW);
      |     if ~strcmp(u16NSamplesW_bkup,tmps)
      |       set_param(gcb,'u16NSamplesW',tmps);
      |     end
      |   end
      |   if isnan(u16NSamplesFW)
      |     if ~strcmp(u16NSamplesFW_bkup,'0')
      |       set_param(gcb,'u16NSamplesFW','0');
      |     end
      |   else
      |     tmps=num2str(u16NSamplesFW);
      |     if ~strcmp(u16NSamplesFW_bkup,tmps)
      |       set_param(gcb,'u16NSamplesFW',tmps);
      |     end
      |   end
      |   if isnan(f32PropGainQ)
      |     if ~strcmp(f32PropGainQ_bkup,'0')
      |       set_param(gcb,'f32PropGainQ','0');
      |     end
      |   else
      |     tmps=num2str(f32PropGainQ);
      |     if ~strcmp(f32PropGainQ_bkup,tmps)
      |       set_param(gcb,'f32PropGainQ',tmps);
      |     end
      |   end
      |   if isnan(f32IntegGainQ)
      |     if ~strcmp(f32IntegGainQ_bkup,'0')
      |       set_param(gcb,'f32IntegGainQ','0');
      |     end
      |   else
      |     tmps=num2str(f32IntegGainQ);
      |     if ~strcmp(f32IntegGainQ_bkup,tmps)
      |       set_param(gcb,'f32IntegGainQ',tmps);
      |     end
      |   end
      |   if isnan(s16PropGainShiftQ)
      |     if ~strcmp(s16PropGainShiftQ_bkup,'0')
      |       set_param(gcb,'s16PropGainShiftQ','0');
      |     end
      |   else
      |     tmps=num2str(s16PropGainShiftQ);
      |     if ~strcmp(s16PropGainShiftQ_bkup,tmps)
      |       set_param(gcb,'s16PropGainShiftQ',tmps);
      |     end
      |   end
      |   if isnan(s16IntegGainShiftQ)
      |     if ~strcmp(s16IntegGainShiftQ_bkup,'0')
      |       set_param(gcb,'s16IntegGainShiftQ','0');
      |     end
      |   else
      |     tmps=num2str(s16IntegGainShiftQ);
      |     if ~strcmp(s16IntegGainShiftQ_bkup,tmps)
      |       set_param(gcb,'s16IntegGainShiftQ',tmps);
      |     end
      |   end
      |   if isnan(f32LowerLimitQ)
      |     if ~strcmp(f32LowerLimitQ_bkup,'0')
      |       set_param(gcb,'f32LowerLimitQ','0');
      |     end
      |   else
      |     tmps=num2str(f32LowerLimitQ);
      |     if ~strcmp(f32LowerLimitQ_bkup,tmps)
      |       set_param(gcb,'f32LowerLimitQ',tmps);
      |     end
      |   end
      |   if isnan(f32UpperLimitQ)
      |     if ~strcmp(f32UpperLimitQ_bkup,'0')
      |       set_param(gcb,'f32UpperLimitQ','0');
      |     end
      |   else
      |     tmps=num2str(f32UpperLimitQ);
      |     if ~strcmp(f32UpperLimitQ_bkup,tmps)
      |       set_param(gcb,'f32UpperLimitQ',tmps);
      |     end
      |   end
      |   if isnan(f32PropGainFW)
      |     if ~strcmp(f32PropGainFW_bkup,'0')
      |       set_param(gcb,'f32PropGainFW','0');
      |     end
      |   else
      |     tmps=num2str(f32PropGainFW);
      |     if ~strcmp(f32PropGainFW_bkup,tmps)
      |       set_param(gcb,'f32PropGainFW',tmps);
      |     end
      |   end
      |   if isnan(f32IntegGainFW)
      |     if ~strcmp(f32IntegGainFW_bkup,'0')
      |       set_param(gcb,'f32IntegGainFW','0');
      |     end
      |   else
      |     tmps=num2str(f32IntegGainFW);
      |     if ~strcmp(f32IntegGainFW_bkup,tmps)
      |       set_param(gcb,'f32IntegGainFW',tmps);
      |     end
      |   end
      |   if isnan(s16PropGainShiftFW)
      |     if ~strcmp(s16PropGainShiftFW_bkup,'0')
      |       set_param(gcb,'s16PropGainShiftFW','0');
      |     end
      |   else
      |     tmps=num2str(s16PropGainShiftFW);
      |     if ~strcmp(s16PropGainShiftFW_bkup,tmps)
      |       set_param(gcb,'s16PropGainShiftFW',tmps);
      |     end
      |   end
      |   if isnan(s16IntegGainShiftFW)
      |     if ~strcmp(s16IntegGainShiftFW_bkup,'0')
      |       set_param(gcb,'s16IntegGainShiftFW','0');
      |     end
      |   else
      |     tmps=num2str(s16IntegGainShiftFW);
      |     if ~strcmp(s16IntegGainShiftFW_bkup,tmps)
      |       set_param(gcb,'s16IntegGainShiftFW',tmps);
      |     end
      |   end
      |   if isnan(f32LowerLimitFW)
      |     if ~strcmp(f32LowerLimitFW_bkup,'0')
      |       set_param(gcb,'f32LowerLimitFW','0');
      |     end
      |   else
      |     tmps=num2str(f32LowerLimitFW);
      |     if ~strcmp(f32LowerLimitFW_bkup,tmps)
      |       set_param(gcb,'f32LowerLimitFW',tmps);
      |     end
      |   end
      |   if isnan(f32UpperLimitFW)
      |     if ~strcmp(f32UpperLimitFW_bkup,'0')
      |       set_param(gcb,'f32UpperLimitFW','0');
      |     end
      |   else
      |     tmps=num2str(f32UpperLimitFW);
      |     if ~strcmp(f32UpperLimitFW_bkup,tmps)
      |       set_param(gcb,'f32UpperLimitFW',tmps);
      |     end
      |   end
      |   if isnan(f32RampUp)
      |     if ~strcmp(f32RampUp_bkup,'0')
      |       set_param(gcb,'f32RampUp','0');
      |     end
      |   else
      |     tmps=num2str(f32RampUp);
      |     if ~strcmp(f32RampUp_bkup,tmps)
      |       set_param(gcb,'f32RampUp',tmps);
      |     end
      |   end
      |   if isnan(f32RampDown)
      |     if ~strcmp(f32RampDown_bkup,'0')
      |       set_param(gcb,'f32RampDown','0');
      |     end
      |   else
      |     tmps=num2str(f32RampDown);
      |     if ~strcmp(f32RampDown_bkup,tmps)
      |       set_param(gcb,'f32RampDown',tmps);
      |     end
      |   end
      | end
      mask Callback lambdaFW:
      | autoCalcEn=get_param(gcb,'autoCalcEn');
      | if strcmp(autoCalcEn,'on')
      |   SampleTime=Simulink.data.evalinGlobal(bdroot,get_param(gcb,'SampleTime'));
      |   if (SampleTime==-1)
      |     SampleTime=str2double(get_param(gcb,'SampleTime_1'));
      |   end
      |   u16NSamplesW_bkup=get_param(gcb,'u16NSamplesW');
      |   u16NSamplesFW_bkup=get_param(gcb,'u16NSamplesFW');
      |   f32PropGainQ_bkup=get_param(gcb,'f32PropGainQ');
      |   f32IntegGainQ_bkup=get_param(gcb,'f32IntegGainQ');
      |   s16PropGainShiftQ_bkup=get_param(gcb,'s16PropGainShiftQ');
      |   s16IntegGainShiftQ_bkup=get_param(gcb,'s16IntegGainShiftQ');
      |   f32LowerLimitQ_bkup=get_param(gcb,'f32LowerLimitQ');
      |   f32UpperLimitQ_bkup=get_param(gcb,'f32UpperLimitQ');
      |   f32PropGainFW_bkup=get_param(gcb,'f32PropGainFW');
      |   f32IntegGainFW_bkup=get_param(gcb,'f32IntegGainFW');
      |   s16PropGainShiftFW_bkup=get_param(gcb,'s16PropGainShiftFW');
      |   s16IntegGainShiftFW_bkup=get_param(gcb,'s16IntegGainShiftFW');
      |   f32LowerLimitFW_bkup=get_param(gcb,'f32LowerLimitFW');
      |   f32UpperLimitFW_bkup=get_param(gcb,'f32UpperLimitFW');
      |   f32RampUp_bkup=get_param(gcb,'f32RampUp');
      |   f32RampDown_bkup=get_param(gcb,'f32RampDown');
      |   wf0=Simulink.data.evalinGlobal(bdroot,get_param(gcb,'wf0'));
      |   wksi=Simulink.data.evalinGlobal(bdroot,get_param(gcb,'wksi'));
      |   J=Simulink.data.evalinGlobal(bdroot,get_param(gcb,'J'));
      |   Kt=Simulink.data.evalinGlobal(bdroot,get_param(gcb,'Kt'));
      |   lambdaW=Simulink.data.evalinGlobal(bdroot,get_param(gcb,'lambdaW'));
      |   lambdaFW=Simulink.data.evalinGlobal(bdroot,get_param(gcb,'lambdaFW'));
      |   Idmax=Simulink.data.evalinGlobal(bdroot,get_param(gcb,'Idmax'));
      |   ramprpm=Simulink.data.evalinGlobal(bdroot,get_param(gcb,'ramprpm'));
      |   mechspeed=Simulink.data.evalinGlobal(bdroot,get_param(gcb,'mechspeed'));
      |   polepairs=Simulink.data.evalinGlobal(bdroot,get_param(gcb,'polepairs'));
      |   uscale=Simulink.data.evalinGlobal(bdroot,get_param(gcb,'uscale'));
      |   iscale=Simulink.data.evalinGlobal(bdroot,get_param(gcb,'iscale'));
      |   if (wf0<=0)
      |     warning('Natural frequency f0 must be positive.');
      |   end
      |   if (wksi<=0)
      |     warning('Current loop attenuation must be positive.');
      |   end
      |   if (wksi>1)
      |     warning('Current loop attenuation must not exceed 1.');
      |   end
      |   if (J<=0)
      |     warning('Moment of inertia J must be positive.');
      |   end
      |   if (Kt<=0)
      |     warning('Torque constant Kt must be positive.');
      |   end
      |   if (lambdaW<0)
      |     warning('MA filter smoothing factor must be in the range 0..1.');
      |   end
      |   if (lambdaW>1)
      |     warning('MA filter smoothing factor must be in the range 0..1.');
      |   end
      |   if (lambdaFW<0)
      |     warning('MA filter smoothing factor must be in the range 0..1.');
      |   end
      |   if (lambdaFW>1)
      |     warning('MA filter smoothing factor must be in the range 0..1.');
      |   end
      |   if (mechspeed<=0)
      |     warning('Max. speed must be positive.');
      |   end
      |   if (polepairs<1)
      |     warning('Number of pole pairs must be a natural number (1, 2, 3, ...).');
      |   end
      |   if (round(polepairs)~=polepairs)
      |     warning('Number of pole pairs must be a natural number (1, 2, 3, ...).');
      |   end
      |   if (uscale<=0)
      |     warning('U_max must be positive.');
      |   end
      |   if (iscale<=0)
      |     warning('I_max must be positive.');
      |   end
      |   w0=6.283185307179586*wf0;
      |   pgain=2.0*wksi*w0*J/Kt;
      |   igain=w0*w0*J/Kt;
      |   wmax=polepairs*mechspeed*0.1047197551196598;
      |   kpf=pgain*wmax/iscale;
      |   s16PropGainShiftQ=ceil(log2(abs(kpf)));
      |   if s16PropGainShiftQ<-31
      |     s16PropGainShiftQ=-31;
      |   end
      |   if s16PropGainShiftQ>31
      |     s16PropGainShiftQ=31;
      |     warning(['Parameter s16PropGainShiftQ of ' gcb ' exceeds the fixed-point range.']);
      |   end
      |   f32PropGainQ=round(kpf*2^(-s16PropGainShiftQ)*2^31);
      |   if f32PropGainQ>2^31-1
      |     f32PropGainQ=2^31-1;
      |     warning(['Parameter f32PropGainQ of ' gcb ' exceeds the fixed-point range.']);
      |   end
      |   if f32PropGainQ<-2^31
      |     f32PropGainQ=-2^31;
      |     warning(['Parameter f32PropGainQ of ' gcb ' exceeds the fixed-point range.']);
      |   end
      |   kif=igain*SampleTime*0.5*wmax/iscale;
      |   s16IntegGainShiftQ=ceil(log2(abs(kif)));
      |   if s16IntegGainShiftQ<-31
      |     s16IntegGainShiftQ=-31;
      |   end
      |   if s16IntegGainShiftQ>31
      |     s16IntegGainShiftQ=31;
      |     warning(['Parameter s16IntegGainShiftQ of ' gcb ' exceeds the fixed-point range.']);
      |   end
      |   f32IntegGainQ=round(kif*2^(-s16IntegGainShiftQ)*2^31);
      |   if f32IntegGainQ>2^31-1
      |     f32IntegGainQ=2^31-1;
      |     warning(['Parameter f32IntegGainQ of ' gcb ' exceeds the fixed-point range.']);
      |   end
      |   if f32IntegGainQ<-2^31
      |     f32IntegGainQ=-2^31;
      |     warning(['Parameter f32IntegGainQ of ' gcb ' exceeds the fixed-point range.']);
      |   end
      |   f32LowerLimitQ=-2147483648;
      |   f32UpperLimitQ=2147483647;
      |   fwkpf=0.9*pgain*wmax/iscale;
      |   s16PropGainShiftFW=ceil(log2(abs(fwkpf)));
      |   if s16PropGainShiftFW<-31
      |     s16PropGainShiftFW=-31;
      |   end
      |   if s16PropGainShiftFW>31
      |     s16PropGainShiftFW=31;
      |     warning(['Parameter s16PropGainShiftFW of ' gcb ' exceeds the fixed-point range.']);
      |   end
      |   f32PropGainFW=round(fwkpf*2^(-s16PropGainShiftFW)*2^31);
      |   if f32PropGainFW>2^31-1
      |     f32PropGainFW=2^31-1;
      |     warning(['Parameter f32PropGainFW of ' gcb ' exceeds the fixed-point range.']);
      |   end
      |   if f32PropGainFW<-2^31
      |     f32PropGainFW=-2^31;
      |     warning(['Parameter f32PropGainFW of ' gcb ' exceeds the fixed-point range.']);
      |   end
      |   s16IntegGainShiftFW=s16IntegGainShiftQ;
      |   f32IntegGainFW=f32IntegGainQ;
      |   if (Idmax<0)
      |     iratio=abs(Idmax)/iscale;
      |     if (abs(iratio) > 1)
      |       iratio = 0;
      |     end
      |     lowlim=0.3183098861837907*acos(iratio)-0.5;
      |   else
      |     lowlim=0.0;
      |   end
      |   f32LowerLimitFW=round(lowlim*2^31);
      |   if f32LowerLimitFW>2^31-1
      |     f32LowerLimitFW=2^31-1;
      |     warning(['Parameter f32LowerLimitFW of ' gcb ' exceeds the fixed-point range.']);
      |   end
      |   if f32LowerLimitFW<-2^31
      |     f32LowerLimitFW=-2^31;
      |     warning(['Parameter f32LowerLimitFW of ' gcb ' exceeds the fixed-point range.']);
      |   end
      |   f32UpperLimitFW=0;
      |   u16NSamplesW=round(log2(1.0/abs(lambdaW)));
      |   if u16NSamplesW>31
      |     u16NSamplesW=31;
      |   end
      |   if u16NSamplesW<0
      |     u16NSamplesW=0;
      |   end
      |   u16NSamplesFW=round(log2(1.0/abs(lambdaFW)));
      |   if u16NSamplesFW>31
      |     u16NSamplesFW=31;
      |   end
      |   if u16NSamplesFW<0
      |     u16NSamplesFW=0;
      |   end
      |   rampsc=polepairs*abs(ramprpm)*0.1047197551196598/wmax;
      |   f32RampUp=round(rampsc*2^31);
      |   if f32RampUp>2^31-1
      |     f32RampUp=2^31-1;
      |     warning(['Parameter f32RampUp of ' gcb ' exceeds the fixed-point range.']);
      |   end
      |   if f32RampUp<-2^31
      |     f32RampUp=-2^31;
      |     warning(['Parameter f32RampUp of ' gcb ' exceeds the fixed-point range.']);
      |   end
      |   f32RampDown=round(rampsc*2^31);
      |   if f32RampDown>2^31-1
      |     f32RampDown=2^31-1;
      |     warning(['Parameter f32RampDown of ' gcb ' exceeds the fixed-point range.']);
      |   end
      |   if f32RampDown<-2^31
      |     f32RampDown=-2^31;
      |     warning(['Parameter f32RampDown of ' gcb ' exceeds the fixed-point range.']);
      |   end
      |   if isnan(u16NSamplesW)
      |     if ~strcmp(u16NSamplesW_bkup,'0')
      |       set_param(gcb,'u16NSamplesW','0');
      |     end
      |   else
      |     tmps=num2str(u16NSamplesW);
      |     if ~strcmp(u16NSamplesW_bkup,tmps)
      |       set_param(gcb,'u16NSamplesW',tmps);
      |     end
      |   end
      |   if isnan(u16NSamplesFW)
      |     if ~strcmp(u16NSamplesFW_bkup,'0')
      |       set_param(gcb,'u16NSamplesFW','0');
      |     end
      |   else
      |     tmps=num2str(u16NSamplesFW);
      |     if ~strcmp(u16NSamplesFW_bkup,tmps)
      |       set_param(gcb,'u16NSamplesFW',tmps);
      |     end
      |   end
      |   if isnan(f32PropGainQ)
      |     if ~strcmp(f32PropGainQ_bkup,'0')
      |       set_param(gcb,'f32PropGainQ','0');
      |     end
      |   else
      |     tmps=num2str(f32PropGainQ);
      |     if ~strcmp(f32PropGainQ_bkup,tmps)
      |       set_param(gcb,'f32PropGainQ',tmps);
      |     end
      |   end
      |   if isnan(f32IntegGainQ)
      |     if ~strcmp(f32IntegGainQ_bkup,'0')
      |       set_param(gcb,'f32IntegGainQ','0');
      |     end
      |   else
      |     tmps=num2str(f32IntegGainQ);
      |     if ~strcmp(f32IntegGainQ_bkup,tmps)
      |       set_param(gcb,'f32IntegGainQ',tmps);
      |     end
      |   end
      |   if isnan(s16PropGainShiftQ)
      |     if ~strcmp(s16PropGainShiftQ_bkup,'0')
      |       set_param(gcb,'s16PropGainShiftQ','0');
      |     end
      |   else
      |     tmps=num2str(s16PropGainShiftQ);
      |     if ~strcmp(s16PropGainShiftQ_bkup,tmps)
      |       set_param(gcb,'s16PropGainShiftQ',tmps);
      |     end
      |   end
      |   if isnan(s16IntegGainShiftQ)
      |     if ~strcmp(s16IntegGainShiftQ_bkup,'0')
      |       set_param(gcb,'s16IntegGainShiftQ','0');
      |     end
      |   else
      |     tmps=num2str(s16IntegGainShiftQ);
      |     if ~strcmp(s16IntegGainShiftQ_bkup,tmps)
      |       set_param(gcb,'s16IntegGainShiftQ',tmps);
      |     end
      |   end
      |   if isnan(f32LowerLimitQ)
      |     if ~strcmp(f32LowerLimitQ_bkup,'0')
      |       set_param(gcb,'f32LowerLimitQ','0');
      |     end
      |   else
      |     tmps=num2str(f32LowerLimitQ);
      |     if ~strcmp(f32LowerLimitQ_bkup,tmps)
      |       set_param(gcb,'f32LowerLimitQ',tmps);
      |     end
      |   end
      |   if isnan(f32UpperLimitQ)
      |     if ~strcmp(f32UpperLimitQ_bkup,'0')
      |       set_param(gcb,'f32UpperLimitQ','0');
      |     end
      |   else
      |     tmps=num2str(f32UpperLimitQ);
      |     if ~strcmp(f32UpperLimitQ_bkup,tmps)
      |       set_param(gcb,'f32UpperLimitQ',tmps);
      |     end
      |   end
      |   if isnan(f32PropGainFW)
      |     if ~strcmp(f32PropGainFW_bkup,'0')
      |       set_param(gcb,'f32PropGainFW','0');
      |     end
      |   else
      |     tmps=num2str(f32PropGainFW);
      |     if ~strcmp(f32PropGainFW_bkup,tmps)
      |       set_param(gcb,'f32PropGainFW',tmps);
      |     end
      |   end
      |   if isnan(f32IntegGainFW)
      |     if ~strcmp(f32IntegGainFW_bkup,'0')
      |       set_param(gcb,'f32IntegGainFW','0');
      |     end
      |   else
      |     tmps=num2str(f32IntegGainFW);
      |     if ~strcmp(f32IntegGainFW_bkup,tmps)
      |       set_param(gcb,'f32IntegGainFW',tmps);
      |     end
      |   end
      |   if isnan(s16PropGainShiftFW)
      |     if ~strcmp(s16PropGainShiftFW_bkup,'0')
      |       set_param(gcb,'s16PropGainShiftFW','0');
      |     end
      |   else
      |     tmps=num2str(s16PropGainShiftFW);
      |     if ~strcmp(s16PropGainShiftFW_bkup,tmps)
      |       set_param(gcb,'s16PropGainShiftFW',tmps);
      |     end
      |   end
      |   if isnan(s16IntegGainShiftFW)
      |     if ~strcmp(s16IntegGainShiftFW_bkup,'0')
      |       set_param(gcb,'s16IntegGainShiftFW','0');
      |     end
      |   else
      |     tmps=num2str(s16IntegGainShiftFW);
      |     if ~strcmp(s16IntegGainShiftFW_bkup,tmps)
      |       set_param(gcb,'s16IntegGainShiftFW',tmps);
      |     end
      |   end
      |   if isnan(f32LowerLimitFW)
      |     if ~strcmp(f32LowerLimitFW_bkup,'0')
      |       set_param(gcb,'f32LowerLimitFW','0');
      |     end
      |   else
      |     tmps=num2str(f32LowerLimitFW);
      |     if ~strcmp(f32LowerLimitFW_bkup,tmps)
      |       set_param(gcb,'f32LowerLimitFW',tmps);
      |     end
      |   end
      |   if isnan(f32UpperLimitFW)
      |     if ~strcmp(f32UpperLimitFW_bkup,'0')
      |       set_param(gcb,'f32UpperLimitFW','0');
      |     end
      |   else
      |     tmps=num2str(f32UpperLimitFW);
      |     if ~strcmp(f32UpperLimitFW_bkup,tmps)
      |       set_param(gcb,'f32UpperLimitFW',tmps);
      |     end
      |   end
      |   if isnan(f32RampUp)
      |     if ~strcmp(f32RampUp_bkup,'0')
      |       set_param(gcb,'f32RampUp','0');
      |     end
      |   else
      |     tmps=num2str(f32RampUp);
      |     if ~strcmp(f32RampUp_bkup,tmps)
      |       set_param(gcb,'f32RampUp',tmps);
      |     end
      |   end
      |   if isnan(f32RampDown)
      |     if ~strcmp(f32RampDown_bkup,'0')
      |       set_param(gcb,'f32RampDown','0');
      |     end
      |   else
      |     tmps=num2str(f32RampDown);
      |     if ~strcmp(f32RampDown_bkup,tmps)
      |       set_param(gcb,'f32RampDown',tmps);
      |     end
      |   end
      | end
      mask Callback Idmax:
      | autoCalcEn=get_param(gcb,'autoCalcEn');
      | if strcmp(autoCalcEn,'on')
      |   SampleTime=Simulink.data.evalinGlobal(bdroot,get_param(gcb,'SampleTime'));
      |   if (SampleTime==-1)
      |     SampleTime=str2double(get_param(gcb,'SampleTime_1'));
      |   end
      |   u16NSamplesW_bkup=get_param(gcb,'u16NSamplesW');
      |   u16NSamplesFW_bkup=get_param(gcb,'u16NSamplesFW');
      |   f32PropGainQ_bkup=get_param(gcb,'f32PropGainQ');
      |   f32IntegGainQ_bkup=get_param(gcb,'f32IntegGainQ');
      |   s16PropGainShiftQ_bkup=get_param(gcb,'s16PropGainShiftQ');
      |   s16IntegGainShiftQ_bkup=get_param(gcb,'s16IntegGainShiftQ');
      |   f32LowerLimitQ_bkup=get_param(gcb,'f32LowerLimitQ');
      |   f32UpperLimitQ_bkup=get_param(gcb,'f32UpperLimitQ');
      |   f32PropGainFW_bkup=get_param(gcb,'f32PropGainFW');
      |   f32IntegGainFW_bkup=get_param(gcb,'f32IntegGainFW');
      |   s16PropGainShiftFW_bkup=get_param(gcb,'s16PropGainShiftFW');
      |   s16IntegGainShiftFW_bkup=get_param(gcb,'s16IntegGainShiftFW');
      |   f32LowerLimitFW_bkup=get_param(gcb,'f32LowerLimitFW');
      |   f32UpperLimitFW_bkup=get_param(gcb,'f32UpperLimitFW');
      |   f32RampUp_bkup=get_param(gcb,'f32RampUp');
      |   f32RampDown_bkup=get_param(gcb,'f32RampDown');
      |   wf0=Simulink.data.evalinGlobal(bdroot,get_param(gcb,'wf0'));
      |   wksi=Simulink.data.evalinGlobal(bdroot,get_param(gcb,'wksi'));
      |   J=Simulink.data.evalinGlobal(bdroot,get_param(gcb,'J'));
      |   Kt=Simulink.data.evalinGlobal(bdroot,get_param(gcb,'Kt'));
      |   lambdaW=Simulink.data.evalinGlobal(bdroot,get_param(gcb,'lambdaW'));
      |   lambdaFW=Simulink.data.evalinGlobal(bdroot,get_param(gcb,'lambdaFW'));
      |   Idmax=Simulink.data.evalinGlobal(bdroot,get_param(gcb,'Idmax'));
      |   ramprpm=Simulink.data.evalinGlobal(bdroot,get_param(gcb,'ramprpm'));
      |   mechspeed=Simulink.data.evalinGlobal(bdroot,get_param(gcb,'mechspeed'));
      |   polepairs=Simulink.data.evalinGlobal(bdroot,get_param(gcb,'polepairs'));
      |   uscale=Simulink.data.evalinGlobal(bdroot,get_param(gcb,'uscale'));
      |   iscale=Simulink.data.evalinGlobal(bdroot,get_param(gcb,'iscale'));
      |   if (wf0<=0)
      |     warning('Natural frequency f0 must be positive.');
      |   end
      |   if (wksi<=0)
      |     warning('Current loop attenuation must be positive.');
      |   end
      |   if (wksi>1)
      |     warning('Current loop attenuation must not exceed 1.');
      |   end
      |   if (J<=0)
      |     warning('Moment of inertia J must be positive.');
      |   end
      |   if (Kt<=0)
      |     warning('Torque constant Kt must be positive.');
      |   end
      |   if (lambdaW<0)
      |     warning('MA filter smoothing factor must be in the range 0..1.');
      |   end
      |   if (lambdaW>1)
      |     warning('MA filter smoothing factor must be in the range 0..1.');
      |   end
      |   if (lambdaFW<0)
      |     warning('MA filter smoothing factor must be in the range 0..1.');
      |   end
      |   if (lambdaFW>1)
      |     warning('MA filter smoothing factor must be in the range 0..1.');
      |   end
      |   if (mechspeed<=0)
      |     warning('Max. speed must be positive.');
      |   end
      |   if (polepairs<1)
      |     warning('Number of pole pairs must be a natural number (1, 2, 3, ...).');
      |   end
      |   if (round(polepairs)~=polepairs)
      |     warning('Number of pole pairs must be a natural number (1, 2, 3, ...).');
      |   end
      |   if (uscale<=0)
      |     warning('U_max must be positive.');
      |   end
      |   if (iscale<=0)
      |     warning('I_max must be positive.');
      |   end
      |   w0=6.283185307179586*wf0;
      |   pgain=2.0*wksi*w0*J/Kt;
      |   igain=w0*w0*J/Kt;
      |   wmax=polepairs*mechspeed*0.1047197551196598;
      |   kpf=pgain*wmax/iscale;
      |   s16PropGainShiftQ=ceil(log2(abs(kpf)));
      |   if s16PropGainShiftQ<-31
      |     s16PropGainShiftQ=-31;
      |   end
      |   if s16PropGainShiftQ>31
      |     s16PropGainShiftQ=31;
      |     warning(['Parameter s16PropGainShiftQ of ' gcb ' exceeds the fixed-point range.']);
      |   end
      |   f32PropGainQ=round(kpf*2^(-s16PropGainShiftQ)*2^31);
      |   if f32PropGainQ>2^31-1
      |     f32PropGainQ=2^31-1;
      |     warning(['Parameter f32PropGainQ of ' gcb ' exceeds the fixed-point range.']);
      |   end
      |   if f32PropGainQ<-2^31
      |     f32PropGainQ=-2^31;
      |     warning(['Parameter f32PropGainQ of ' gcb ' exceeds the fixed-point range.']);
      |   end
      |   kif=igain*SampleTime*0.5*wmax/iscale;
      |   s16IntegGainShiftQ=ceil(log2(abs(kif)));
      |   if s16IntegGainShiftQ<-31
      |     s16IntegGainShiftQ=-31;
      |   end
      |   if s16IntegGainShiftQ>31
      |     s16IntegGainShiftQ=31;
      |     warning(['Parameter s16IntegGainShiftQ of ' gcb ' exceeds the fixed-point range.']);
      |   end
      |   f32IntegGainQ=round(kif*2^(-s16IntegGainShiftQ)*2^31);
      |   if f32IntegGainQ>2^31-1
      |     f32IntegGainQ=2^31-1;
      |     warning(['Parameter f32IntegGainQ of ' gcb ' exceeds the fixed-point range.']);
      |   end
      |   if f32IntegGainQ<-2^31
      |     f32IntegGainQ=-2^31;
      |     warning(['Parameter f32IntegGainQ of ' gcb ' exceeds the fixed-point range.']);
      |   end
      |   f32LowerLimitQ=-2147483648;
      |   f32UpperLimitQ=2147483647;
      |   fwkpf=0.9*pgain*wmax/iscale;
      |   s16PropGainShiftFW=ceil(log2(abs(fwkpf)));
      |   if s16PropGainShiftFW<-31
      |     s16PropGainShiftFW=-31;
      |   end
      |   if s16PropGainShiftFW>31
      |     s16PropGainShiftFW=31;
      |     warning(['Parameter s16PropGainShiftFW of ' gcb ' exceeds the fixed-point range.']);
      |   end
      |   f32PropGainFW=round(fwkpf*2^(-s16PropGainShiftFW)*2^31);
      |   if f32PropGainFW>2^31-1
      |     f32PropGainFW=2^31-1;
      |     warning(['Parameter f32PropGainFW of ' gcb ' exceeds the fixed-point range.']);
      |   end
      |   if f32PropGainFW<-2^31
      |     f32PropGainFW=-2^31;
      |     warning(['Parameter f32PropGainFW of ' gcb ' exceeds the fixed-point range.']);
      |   end
      |   s16IntegGainShiftFW=s16IntegGainShiftQ;
      |   f32IntegGainFW=f32IntegGainQ;
      |   if (Idmax<0)
      |     iratio=abs(Idmax)/iscale;
      |     if (abs(iratio) > 1)
      |       iratio = 0;
      |     end
      |     lowlim=0.3183098861837907*acos(iratio)-0.5;
      |   else
      |     lowlim=0.0;
      |   end
      |   f32LowerLimitFW=round(lowlim*2^31);
      |   if f32LowerLimitFW>2^31-1
      |     f32LowerLimitFW=2^31-1;
      |     warning(['Parameter f32LowerLimitFW of ' gcb ' exceeds the fixed-point range.']);
      |   end
      |   if f32LowerLimitFW<-2^31
      |     f32LowerLimitFW=-2^31;
      |     warning(['Parameter f32LowerLimitFW of ' gcb ' exceeds the fixed-point range.']);
      |   end
      |   f32UpperLimitFW=0;
      |   u16NSamplesW=round(log2(1.0/abs(lambdaW)));
      |   if u16NSamplesW>31
      |     u16NSamplesW=31;
      |   end
      |   if u16NSamplesW<0
      |     u16NSamplesW=0;
      |   end
      |   u16NSamplesFW=round(log2(1.0/abs(lambdaFW)));
      |   if u16NSamplesFW>31
      |     u16NSamplesFW=31;
      |   end
      |   if u16NSamplesFW<0
      |     u16NSamplesFW=0;
      |   end
      |   rampsc=polepairs*abs(ramprpm)*0.1047197551196598/wmax;
      |   f32RampUp=round(rampsc*2^31);
      |   if f32RampUp>2^31-1
      |     f32RampUp=2^31-1;
      |     warning(['Parameter f32RampUp of ' gcb ' exceeds the fixed-point range.']);
      |   end
      |   if f32RampUp<-2^31
      |     f32RampUp=-2^31;
      |     warning(['Parameter f32RampUp of ' gcb ' exceeds the fixed-point range.']);
      |   end
      |   f32RampDown=round(rampsc*2^31);
      |   if f32RampDown>2^31-1
      |     f32RampDown=2^31-1;
      |     warning(['Parameter f32RampDown of ' gcb ' exceeds the fixed-point range.']);
      |   end
      |   if f32RampDown<-2^31
      |     f32RampDown=-2^31;
      |     warning(['Parameter f32RampDown of ' gcb ' exceeds the fixed-point range.']);
      |   end
      |   if isnan(u16NSamplesW)
      |     if ~strcmp(u16NSamplesW_bkup,'0')
      |       set_param(gcb,'u16NSamplesW','0');
      |     end
      |   else
      |     tmps=num2str(u16NSamplesW);
      |     if ~strcmp(u16NSamplesW_bkup,tmps)
      |       set_param(gcb,'u16NSamplesW',tmps);
      |     end
      |   end
      |   if isnan(u16NSamplesFW)
      |     if ~strcmp(u16NSamplesFW_bkup,'0')
      |       set_param(gcb,'u16NSamplesFW','0');
      |     end
      |   else
      |     tmps=num2str(u16NSamplesFW);
      |     if ~strcmp(u16NSamplesFW_bkup,tmps)
      |       set_param(gcb,'u16NSamplesFW',tmps);
      |     end
      |   end
      |   if isnan(f32PropGainQ)
      |     if ~strcmp(f32PropGainQ_bkup,'0')
      |       set_param(gcb,'f32PropGainQ','0');
      |     end
      |   else
      |     tmps=num2str(f32PropGainQ);
      |     if ~strcmp(f32PropGainQ_bkup,tmps)
      |       set_param(gcb,'f32PropGainQ',tmps);
      |     end
      |   end
      |   if isnan(f32IntegGainQ)
      |     if ~strcmp(f32IntegGainQ_bkup,'0')
      |       set_param(gcb,'f32IntegGainQ','0');
      |     end
      |   else
      |     tmps=num2str(f32IntegGainQ);
      |     if ~strcmp(f32IntegGainQ_bkup,tmps)
      |       set_param(gcb,'f32IntegGainQ',tmps);
      |     end
      |   end
      |   if isnan(s16PropGainShiftQ)
      |     if ~strcmp(s16PropGainShiftQ_bkup,'0')
      |       set_param(gcb,'s16PropGainShiftQ','0');
      |     end
      |   else
      |     tmps=num2str(s16PropGainShiftQ);
      |     if ~strcmp(s16PropGainShiftQ_bkup,tmps)
      |       set_param(gcb,'s16PropGainShiftQ',tmps);
      |     end
      |   end
      |   if isnan(s16IntegGainShiftQ)
      |     if ~strcmp(s16IntegGainShiftQ_bkup,'0')
      |       set_param(gcb,'s16IntegGainShiftQ','0');
      |     end
      |   else
      |     tmps=num2str(s16IntegGainShiftQ);
      |     if ~strcmp(s16IntegGainShiftQ_bkup,tmps)
      |       set_param(gcb,'s16IntegGainShiftQ',tmps);
      |     end
      |   end
      |   if isnan(f32LowerLimitQ)
      |     if ~strcmp(f32LowerLimitQ_bkup,'0')
      |       set_param(gcb,'f32LowerLimitQ','0');
      |     end
      |   else
      |     tmps=num2str(f32LowerLimitQ);
      |     if ~strcmp(f32LowerLimitQ_bkup,tmps)
      |       set_param(gcb,'f32LowerLimitQ',tmps);
      |     end
      |   end
      |   if isnan(f32UpperLimitQ)
      |     if ~strcmp(f32UpperLimitQ_bkup,'0')
      |       set_param(gcb,'f32UpperLimitQ','0');
      |     end
      |   else
      |     tmps=num2str(f32UpperLimitQ);
      |     if ~strcmp(f32UpperLimitQ_bkup,tmps)
      |       set_param(gcb,'f32UpperLimitQ',tmps);
      |     end
      |   end
      |   if isnan(f32PropGainFW)
      |     if ~strcmp(f32PropGainFW_bkup,'0')
      |       set_param(gcb,'f32PropGainFW','0');
      |     end
      |   else
      |     tmps=num2str(f32PropGainFW);
      |     if ~strcmp(f32PropGainFW_bkup,tmps)
      |       set_param(gcb,'f32PropGainFW',tmps);
      |     end
      |   end
      |   if isnan(f32IntegGainFW)
      |     if ~strcmp(f32IntegGainFW_bkup,'0')
      |       set_param(gcb,'f32IntegGainFW','0');
      |     end
      |   else
      |     tmps=num2str(f32IntegGainFW);
      |     if ~strcmp(f32IntegGainFW_bkup,tmps)
      |       set_param(gcb,'f32IntegGainFW',tmps);
      |     end
      |   end
      |   if isnan(s16PropGainShiftFW)
      |     if ~strcmp(s16PropGainShiftFW_bkup,'0')
      |       set_param(gcb,'s16PropGainShiftFW','0');
      |     end
      |   else
      |     tmps=num2str(s16PropGainShiftFW);
      |     if ~strcmp(s16PropGainShiftFW_bkup,tmps)
      |       set_param(gcb,'s16PropGainShiftFW',tmps);
      |     end
      |   end
      |   if isnan(s16IntegGainShiftFW)
      |     if ~strcmp(s16IntegGainShiftFW_bkup,'0')
      |       set_param(gcb,'s16IntegGainShiftFW','0');
      |     end
      |   else
      |     tmps=num2str(s16IntegGainShiftFW);
      |     if ~strcmp(s16IntegGainShiftFW_bkup,tmps)
      |       set_param(gcb,'s16IntegGainShiftFW',tmps);
      |     end
      |   end
      |   if isnan(f32LowerLimitFW)
      |     if ~strcmp(f32LowerLimitFW_bkup,'0')
      |       set_param(gcb,'f32LowerLimitFW','0');
      |     end
      |   else
      |     tmps=num2str(f32LowerLimitFW);
      |     if ~strcmp(f32LowerLimitFW_bkup,tmps)
      |       set_param(gcb,'f32LowerLimitFW',tmps);
      |     end
      |   end
      |   if isnan(f32UpperLimitFW)
      |     if ~strcmp(f32UpperLimitFW_bkup,'0')
      |       set_param(gcb,'f32UpperLimitFW','0');
      |     end
      |   else
      |     tmps=num2str(f32UpperLimitFW);
      |     if ~strcmp(f32UpperLimitFW_bkup,tmps)
      |       set_param(gcb,'f32UpperLimitFW',tmps);
      |     end
      |   end
      |   if isnan(f32RampUp)
      |     if ~strcmp(f32RampUp_bkup,'0')
      |       set_param(gcb,'f32RampUp','0');
      |     end
      |   else
      |     tmps=num2str(f32RampUp);
      |     if ~strcmp(f32RampUp_bkup,tmps)
      |       set_param(gcb,'f32RampUp',tmps);
      |     end
      |   end
      |   if isnan(f32RampDown)
      |     if ~strcmp(f32RampDown_bkup,'0')
      |       set_param(gcb,'f32RampDown','0');
      |     end
      |   else
      |     tmps=num2str(f32RampDown);
      |     if ~strcmp(f32RampDown_bkup,tmps)
      |       set_param(gcb,'f32RampDown',tmps);
      |     end
      |   end
      | end
      mask Callback ramprpm:
      | autoCalcEn=get_param(gcb,'autoCalcEn');
      | if strcmp(autoCalcEn,'on')
      |   SampleTime=Simulink.data.evalinGlobal(bdroot,get_param(gcb,'SampleTime'));
      |   if (SampleTime==-1)
      |     SampleTime=str2double(get_param(gcb,'SampleTime_1'));
      |   end
      |   u16NSamplesW_bkup=get_param(gcb,'u16NSamplesW');
      |   u16NSamplesFW_bkup=get_param(gcb,'u16NSamplesFW');
      |   f32PropGainQ_bkup=get_param(gcb,'f32PropGainQ');
      |   f32IntegGainQ_bkup=get_param(gcb,'f32IntegGainQ');
      |   s16PropGainShiftQ_bkup=get_param(gcb,'s16PropGainShiftQ');
      |   s16IntegGainShiftQ_bkup=get_param(gcb,'s16IntegGainShiftQ');
      |   f32LowerLimitQ_bkup=get_param(gcb,'f32LowerLimitQ');
      |   f32UpperLimitQ_bkup=get_param(gcb,'f32UpperLimitQ');
      |   f32PropGainFW_bkup=get_param(gcb,'f32PropGainFW');
      |   f32IntegGainFW_bkup=get_param(gcb,'f32IntegGainFW');
      |   s16PropGainShiftFW_bkup=get_param(gcb,'s16PropGainShiftFW');
      |   s16IntegGainShiftFW_bkup=get_param(gcb,'s16IntegGainShiftFW');
      |   f32LowerLimitFW_bkup=get_param(gcb,'f32LowerLimitFW');
      |   f32UpperLimitFW_bkup=get_param(gcb,'f32UpperLimitFW');
      |   f32RampUp_bkup=get_param(gcb,'f32RampUp');
      |   f32RampDown_bkup=get_param(gcb,'f32RampDown');
      |   wf0=Simulink.data.evalinGlobal(bdroot,get_param(gcb,'wf0'));
      |   wksi=Simulink.data.evalinGlobal(bdroot,get_param(gcb,'wksi'));
      |   J=Simulink.data.evalinGlobal(bdroot,get_param(gcb,'J'));
      |   Kt=Simulink.data.evalinGlobal(bdroot,get_param(gcb,'Kt'));
      |   lambdaW=Simulink.data.evalinGlobal(bdroot,get_param(gcb,'lambdaW'));
      |   lambdaFW=Simulink.data.evalinGlobal(bdroot,get_param(gcb,'lambdaFW'));
      |   Idmax=Simulink.data.evalinGlobal(bdroot,get_param(gcb,'Idmax'));
      |   ramprpm=Simulink.data.evalinGlobal(bdroot,get_param(gcb,'ramprpm'));
      |   mechspeed=Simulink.data.evalinGlobal(bdroot,get_param(gcb,'mechspeed'));
      |   polepairs=Simulink.data.evalinGlobal(bdroot,get_param(gcb,'polepairs'));
      |   uscale=Simulink.data.evalinGlobal(bdroot,get_param(gcb,'uscale'));
      |   iscale=Simulink.data.evalinGlobal(bdroot,get_param(gcb,'iscale'));
      |   if (wf0<=0)
      |     warning('Natural frequency f0 must be positive.');
      |   end
      |   if (wksi<=0)
      |     warning('Current loop attenuation must be positive.');
      |   end
      |   if (wksi>1)
      |     warning('Current loop attenuation must not exceed 1.');
      |   end
      |   if (J<=0)
      |     warning('Moment of inertia J must be positive.');
      |   end
      |   if (Kt<=0)
      |     warning('Torque constant Kt must be positive.');
      |   end
      |   if (lambdaW<0)
      |     warning('MA filter smoothing factor must be in the range 0..1.');
      |   end
      |   if (lambdaW>1)
      |     warning('MA filter smoothing factor must be in the range 0..1.');
      |   end
      |   if (lambdaFW<0)
      |     warning('MA filter smoothing factor must be in the range 0..1.');
      |   end
      |   if (lambdaFW>1)
      |     warning('MA filter smoothing factor must be in the range 0..1.');
      |   end
      |   if (mechspeed<=0)
      |     warning('Max. speed must be positive.');
      |   end
      |   if (polepairs<1)
      |     warning('Number of pole pairs must be a natural number (1, 2, 3, ...).');
      |   end
      |   if (round(polepairs)~=polepairs)
      |     warning('Number of pole pairs must be a natural number (1, 2, 3, ...).');
      |   end
      |   if (uscale<=0)
      |     warning('U_max must be positive.');
      |   end
      |   if (iscale<=0)
      |     warning('I_max must be positive.');
      |   end
      |   w0=6.283185307179586*wf0;
      |   pgain=2.0*wksi*w0*J/Kt;
      |   igain=w0*w0*J/Kt;
      |   wmax=polepairs*mechspeed*0.1047197551196598;
      |   kpf=pgain*wmax/iscale;
      |   s16PropGainShiftQ=ceil(log2(abs(kpf)));
      |   if s16PropGainShiftQ<-31
      |     s16PropGainShiftQ=-31;
      |   end
      |   if s16PropGainShiftQ>31
      |     s16PropGainShiftQ=31;
      |     warning(['Parameter s16PropGainShiftQ of ' gcb ' exceeds the fixed-point range.']);
      |   end
      |   f32PropGainQ=round(kpf*2^(-s16PropGainShiftQ)*2^31);
      |   if f32PropGainQ>2^31-1
      |     f32PropGainQ=2^31-1;
      |     warning(['Parameter f32PropGainQ of ' gcb ' exceeds the fixed-point range.']);
      |   end
      |   if f32PropGainQ<-2^31
      |     f32PropGainQ=-2^31;
      |     warning(['Parameter f32PropGainQ of ' gcb ' exceeds the fixed-point range.']);
      |   end
      |   kif=igain*SampleTime*0.5*wmax/iscale;
      |   s16IntegGainShiftQ=ceil(log2(abs(kif)));
      |   if s16IntegGainShiftQ<-31
      |     s16IntegGainShiftQ=-31;
      |   end
      |   if s16IntegGainShiftQ>31
      |     s16IntegGainShiftQ=31;
      |     warning(['Parameter s16IntegGainShiftQ of ' gcb ' exceeds the fixed-point range.']);
      |   end
      |   f32IntegGainQ=round(kif*2^(-s16IntegGainShiftQ)*2^31);
      |   if f32IntegGainQ>2^31-1
      |     f32IntegGainQ=2^31-1;
      |     warning(['Parameter f32IntegGainQ of ' gcb ' exceeds the fixed-point range.']);
      |   end
      |   if f32IntegGainQ<-2^31
      |     f32IntegGainQ=-2^31;
      |     warning(['Parameter f32IntegGainQ of ' gcb ' exceeds the fixed-point range.']);
      |   end
      |   f32LowerLimitQ=-2147483648;
      |   f32UpperLimitQ=2147483647;
      |   fwkpf=0.9*pgain*wmax/iscale;
      |   s16PropGainShiftFW=ceil(log2(abs(fwkpf)));
      |   if s16PropGainShiftFW<-31
      |     s16PropGainShiftFW=-31;
      |   end
      |   if s16PropGainShiftFW>31
      |     s16PropGainShiftFW=31;
      |     warning(['Parameter s16PropGainShiftFW of ' gcb ' exceeds the fixed-point range.']);
      |   end
      |   f32PropGainFW=round(fwkpf*2^(-s16PropGainShiftFW)*2^31);
      |   if f32PropGainFW>2^31-1
      |     f32PropGainFW=2^31-1;
      |     warning(['Parameter f32PropGainFW of ' gcb ' exceeds the fixed-point range.']);
      |   end
      |   if f32PropGainFW<-2^31
      |     f32PropGainFW=-2^31;
      |     warning(['Parameter f32PropGainFW of ' gcb ' exceeds the fixed-point range.']);
      |   end
      |   s16IntegGainShiftFW=s16IntegGainShiftQ;
      |   f32IntegGainFW=f32IntegGainQ;
      |   if (Idmax<0)
      |     iratio=abs(Idmax)/iscale;
      |     if (abs(iratio) > 1)
      |       iratio = 0;
      |     end
      |     lowlim=0.3183098861837907*acos(iratio)-0.5;
      |   else
      |     lowlim=0.0;
      |   end
      |   f32LowerLimitFW=round(lowlim*2^31);
      |   if f32LowerLimitFW>2^31-1
      |     f32LowerLimitFW=2^31-1;
      |     warning(['Parameter f32LowerLimitFW of ' gcb ' exceeds the fixed-point range.']);
      |   end
      |   if f32LowerLimitFW<-2^31
      |     f32LowerLimitFW=-2^31;
      |     warning(['Parameter f32LowerLimitFW of ' gcb ' exceeds the fixed-point range.']);
      |   end
      |   f32UpperLimitFW=0;
      |   u16NSamplesW=round(log2(1.0/abs(lambdaW)));
      |   if u16NSamplesW>31
      |     u16NSamplesW=31;
      |   end
      |   if u16NSamplesW<0
      |     u16NSamplesW=0;
      |   end
      |   u16NSamplesFW=round(log2(1.0/abs(lambdaFW)));
      |   if u16NSamplesFW>31
      |     u16NSamplesFW=31;
      |   end
      |   if u16NSamplesFW<0
      |     u16NSamplesFW=0;
      |   end
      |   rampsc=polepairs*abs(ramprpm)*0.1047197551196598/wmax;
      |   f32RampUp=round(rampsc*2^31);
      |   if f32RampUp>2^31-1
      |     f32RampUp=2^31-1;
      |     warning(['Parameter f32RampUp of ' gcb ' exceeds the fixed-point range.']);
      |   end
      |   if f32RampUp<-2^31
      |     f32RampUp=-2^31;
      |     warning(['Parameter f32RampUp of ' gcb ' exceeds the fixed-point range.']);
      |   end
      |   f32RampDown=round(rampsc*2^31);
      |   if f32RampDown>2^31-1
      |     f32RampDown=2^31-1;
      |     warning(['Parameter f32RampDown of ' gcb ' exceeds the fixed-point range.']);
      |   end
      |   if f32RampDown<-2^31
      |     f32RampDown=-2^31;
      |     warning(['Parameter f32RampDown of ' gcb ' exceeds the fixed-point range.']);
      |   end
      |   if isnan(u16NSamplesW)
      |     if ~strcmp(u16NSamplesW_bkup,'0')
      |       set_param(gcb,'u16NSamplesW','0');
      |     end
      |   else
      |     tmps=num2str(u16NSamplesW);
      |     if ~strcmp(u16NSamplesW_bkup,tmps)
      |       set_param(gcb,'u16NSamplesW',tmps);
      |     end
      |   end
      |   if isnan(u16NSamplesFW)
      |     if ~strcmp(u16NSamplesFW_bkup,'0')
      |       set_param(gcb,'u16NSamplesFW','0');
      |     end
      |   else
      |     tmps=num2str(u16NSamplesFW);
      |     if ~strcmp(u16NSamplesFW_bkup,tmps)
      |       set_param(gcb,'u16NSamplesFW',tmps);
      |     end
      |   end
      |   if isnan(f32PropGainQ)
      |     if ~strcmp(f32PropGainQ_bkup,'0')
      |       set_param(gcb,'f32PropGainQ','0');
      |     end
      |   else
      |     tmps=num2str(f32PropGainQ);
      |     if ~strcmp(f32PropGainQ_bkup,tmps)
      |       set_param(gcb,'f32PropGainQ',tmps);
      |     end
      |   end
      |   if isnan(f32IntegGainQ)
      |     if ~strcmp(f32IntegGainQ_bkup,'0')
      |       set_param(gcb,'f32IntegGainQ','0');
      |     end
      |   else
      |     tmps=num2str(f32IntegGainQ);
      |     if ~strcmp(f32IntegGainQ_bkup,tmps)
      |       set_param(gcb,'f32IntegGainQ',tmps);
      |     end
      |   end
      |   if isnan(s16PropGainShiftQ)
      |     if ~strcmp(s16PropGainShiftQ_bkup,'0')
      |       set_param(gcb,'s16PropGainShiftQ','0');
      |     end
      |   else
      |     tmps=num2str(s16PropGainShiftQ);
      |     if ~strcmp(s16PropGainShiftQ_bkup,tmps)
      |       set_param(gcb,'s16PropGainShiftQ',tmps);
      |     end
      |   end
      |   if isnan(s16IntegGainShiftQ)
      |     if ~strcmp(s16IntegGainShiftQ_bkup,'0')
      |       set_param(gcb,'s16IntegGainShiftQ','0');
      |     end
      |   else
      |     tmps=num2str(s16IntegGainShiftQ);
      |     if ~strcmp(s16IntegGainShiftQ_bkup,tmps)
      |       set_param(gcb,'s16IntegGainShiftQ',tmps);
      |     end
      |   end
      |   if isnan(f32LowerLimitQ)
      |     if ~strcmp(f32LowerLimitQ_bkup,'0')
      |       set_param(gcb,'f32LowerLimitQ','0');
      |     end
      |   else
      |     tmps=num2str(f32LowerLimitQ);
      |     if ~strcmp(f32LowerLimitQ_bkup,tmps)
      |       set_param(gcb,'f32LowerLimitQ',tmps);
      |     end
      |   end
      |   if isnan(f32UpperLimitQ)
      |     if ~strcmp(f32UpperLimitQ_bkup,'0')
      |       set_param(gcb,'f32UpperLimitQ','0');
      |     end
      |   else
      |     tmps=num2str(f32UpperLimitQ);
      |     if ~strcmp(f32UpperLimitQ_bkup,tmps)
      |       set_param(gcb,'f32UpperLimitQ',tmps);
      |     end
      |   end
      |   if isnan(f32PropGainFW)
      |     if ~strcmp(f32PropGainFW_bkup,'0')
      |       set_param(gcb,'f32PropGainFW','0');
      |     end
      |   else
      |     tmps=num2str(f32PropGainFW);
      |     if ~strcmp(f32PropGainFW_bkup,tmps)
      |       set_param(gcb,'f32PropGainFW',tmps);
      |     end
      |   end
      |   if isnan(f32IntegGainFW)
      |     if ~strcmp(f32IntegGainFW_bkup,'0')
      |       set_param(gcb,'f32IntegGainFW','0');
      |     end
      |   else
      |     tmps=num2str(f32IntegGainFW);
      |     if ~strcmp(f32IntegGainFW_bkup,tmps)
      |       set_param(gcb,'f32IntegGainFW',tmps);
      |     end
      |   end
      |   if isnan(s16PropGainShiftFW)
      |     if ~strcmp(s16PropGainShiftFW_bkup,'0')
      |       set_param(gcb,'s16PropGainShiftFW','0');
      |     end
      |   else
      |     tmps=num2str(s16PropGainShiftFW);
      |     if ~strcmp(s16PropGainShiftFW_bkup,tmps)
      |       set_param(gcb,'s16PropGainShiftFW',tmps);
      |     end
      |   end
      |   if isnan(s16IntegGainShiftFW)
      |     if ~strcmp(s16IntegGainShiftFW_bkup,'0')
      |       set_param(gcb,'s16IntegGainShiftFW','0');
      |     end
      |   else
      |     tmps=num2str(s16IntegGainShiftFW);
      |     if ~strcmp(s16IntegGainShiftFW_bkup,tmps)
      |       set_param(gcb,'s16IntegGainShiftFW',tmps);
      |     end
      |   end
      |   if isnan(f32LowerLimitFW)
      |     if ~strcmp(f32LowerLimitFW_bkup,'0')
      |       set_param(gcb,'f32LowerLimitFW','0');
      |     end
      |   else
      |     tmps=num2str(f32LowerLimitFW);
      |     if ~strcmp(f32LowerLimitFW_bkup,tmps)
      |       set_param(gcb,'f32LowerLimitFW',tmps);
      |     end
      |   end
      |   if isnan(f32UpperLimitFW)
      |     if ~strcmp(f32UpperLimitFW_bkup,'0')
      |       set_param(gcb,'f32UpperLimitFW','0');
      |     end
      |   else
      |     tmps=num2str(f32UpperLimitFW);
      |     if ~strcmp(f32UpperLimitFW_bkup,tmps)
      |       set_param(gcb,'f32UpperLimitFW',tmps);
      |     end
      |   end
      |   if isnan(f32RampUp)
      |     if ~strcmp(f32RampUp_bkup,'0')
      |       set_param(gcb,'f32RampUp','0');
      |     end
      |   else
      |     tmps=num2str(f32RampUp);
      |     if ~strcmp(f32RampUp_bkup,tmps)
      |       set_param(gcb,'f32RampUp',tmps);
      |     end
      |   end
      |   if isnan(f32RampDown)
      |     if ~strcmp(f32RampDown_bkup,'0')
      |       set_param(gcb,'f32RampDown','0');
      |     end
      |   else
      |     tmps=num2str(f32RampDown);
      |     if ~strcmp(f32RampDown_bkup,tmps)
      |       set_param(gcb,'f32RampDown',tmps);
      |     end
      |   end
      | end
      mask Callback mechspeed:
      | autoCalcEn=get_param(gcb,'autoCalcEn');
      | if strcmp(autoCalcEn,'on')
      |   SampleTime=Simulink.data.evalinGlobal(bdroot,get_param(gcb,'SampleTime'));
      |   if (SampleTime==-1)
      |     SampleTime=str2double(get_param(gcb,'SampleTime_1'));
      |   end
      |   u16NSamplesW_bkup=get_param(gcb,'u16NSamplesW');
      |   u16NSamplesFW_bkup=get_param(gcb,'u16NSamplesFW');
      |   f32PropGainQ_bkup=get_param(gcb,'f32PropGainQ');
      |   f32IntegGainQ_bkup=get_param(gcb,'f32IntegGainQ');
      |   s16PropGainShiftQ_bkup=get_param(gcb,'s16PropGainShiftQ');
      |   s16IntegGainShiftQ_bkup=get_param(gcb,'s16IntegGainShiftQ');
      |   f32LowerLimitQ_bkup=get_param(gcb,'f32LowerLimitQ');
      |   f32UpperLimitQ_bkup=get_param(gcb,'f32UpperLimitQ');
      |   f32PropGainFW_bkup=get_param(gcb,'f32PropGainFW');
      |   f32IntegGainFW_bkup=get_param(gcb,'f32IntegGainFW');
      |   s16PropGainShiftFW_bkup=get_param(gcb,'s16PropGainShiftFW');
      |   s16IntegGainShiftFW_bkup=get_param(gcb,'s16IntegGainShiftFW');
      |   f32LowerLimitFW_bkup=get_param(gcb,'f32LowerLimitFW');
      |   f32UpperLimitFW_bkup=get_param(gcb,'f32UpperLimitFW');
      |   f32RampUp_bkup=get_param(gcb,'f32RampUp');
      |   f32RampDown_bkup=get_param(gcb,'f32RampDown');
      |   wf0=Simulink.data.evalinGlobal(bdroot,get_param(gcb,'wf0'));
      |   wksi=Simulink.data.evalinGlobal(bdroot,get_param(gcb,'wksi'));
      |   J=Simulink.data.evalinGlobal(bdroot,get_param(gcb,'J'));
      |   Kt=Simulink.data.evalinGlobal(bdroot,get_param(gcb,'Kt'));
      |   lambdaW=Simulink.data.evalinGlobal(bdroot,get_param(gcb,'lambdaW'));
      |   lambdaFW=Simulink.data.evalinGlobal(bdroot,get_param(gcb,'lambdaFW'));
      |   Idmax=Simulink.data.evalinGlobal(bdroot,get_param(gcb,'Idmax'));
      |   ramprpm=Simulink.data.evalinGlobal(bdroot,get_param(gcb,'ramprpm'));
      |   mechspeed=Simulink.data.evalinGlobal(bdroot,get_param(gcb,'mechspeed'));
      |   polepairs=Simulink.data.evalinGlobal(bdroot,get_param(gcb,'polepairs'));
      |   uscale=Simulink.data.evalinGlobal(bdroot,get_param(gcb,'uscale'));
      |   iscale=Simulink.data.evalinGlobal(bdroot,get_param(gcb,'iscale'));
      |   if (wf0<=0)
      |     warning('Natural frequency f0 must be positive.');
      |   end
      |   if (wksi<=0)
      |     warning('Current loop attenuation must be positive.');
      |   end
      |   if (wksi>1)
      |     warning('Current loop attenuation must not exceed 1.');
      |   end
      |   if (J<=0)
      |     warning('Moment of inertia J must be positive.');
      |   end
      |   if (Kt<=0)
      |     warning('Torque constant Kt must be positive.');
      |   end
      |   if (lambdaW<0)
      |     warning('MA filter smoothing factor must be in the range 0..1.');
      |   end
      |   if (lambdaW>1)
      |     warning('MA filter smoothing factor must be in the range 0..1.');
      |   end
      |   if (lambdaFW<0)
      |     warning('MA filter smoothing factor must be in the range 0..1.');
      |   end
      |   if (lambdaFW>1)
      |     warning('MA filter smoothing factor must be in the range 0..1.');
      |   end
      |   if (mechspeed<=0)
      |     warning('Max. speed must be positive.');
      |   end
      |   if (polepairs<1)
      |     warning('Number of pole pairs must be a natural number (1, 2, 3, ...).');
      |   end
      |   if (round(polepairs)~=polepairs)
      |     warning('Number of pole pairs must be a natural number (1, 2, 3, ...).');
      |   end
      |   if (uscale<=0)
      |     warning('U_max must be positive.');
      |   end
      |   if (iscale<=0)
      |     warning('I_max must be positive.');
      |   end
      |   w0=6.283185307179586*wf0;
      |   pgain=2.0*wksi*w0*J/Kt;
      |   igain=w0*w0*J/Kt;
      |   wmax=polepairs*mechspeed*0.1047197551196598;
      |   kpf=pgain*wmax/iscale;
      |   s16PropGainShiftQ=ceil(log2(abs(kpf)));
      |   if s16PropGainShiftQ<-31
      |     s16PropGainShiftQ=-31;
      |   end
      |   if s16PropGainShiftQ>31
      |     s16PropGainShiftQ=31;
      |     warning(['Parameter s16PropGainShiftQ of ' gcb ' exceeds the fixed-point range.']);
      |   end
      |   f32PropGainQ=round(kpf*2^(-s16PropGainShiftQ)*2^31);
      |   if f32PropGainQ>2^31-1
      |     f32PropGainQ=2^31-1;
      |     warning(['Parameter f32PropGainQ of ' gcb ' exceeds the fixed-point range.']);
      |   end
      |   if f32PropGainQ<-2^31
      |     f32PropGainQ=-2^31;
      |     warning(['Parameter f32PropGainQ of ' gcb ' exceeds the fixed-point range.']);
      |   end
      |   kif=igain*SampleTime*0.5*wmax/iscale;
      |   s16IntegGainShiftQ=ceil(log2(abs(kif)));
      |   if s16IntegGainShiftQ<-31
      |     s16IntegGainShiftQ=-31;
      |   end
      |   if s16IntegGainShiftQ>31
      |     s16IntegGainShiftQ=31;
      |     warning(['Parameter s16IntegGainShiftQ of ' gcb ' exceeds the fixed-point range.']);
      |   end
      |   f32IntegGainQ=round(kif*2^(-s16IntegGainShiftQ)*2^31);
      |   if f32IntegGainQ>2^31-1
      |     f32IntegGainQ=2^31-1;
      |     warning(['Parameter f32IntegGainQ of ' gcb ' exceeds the fixed-point range.']);
      |   end
      |   if f32IntegGainQ<-2^31
      |     f32IntegGainQ=-2^31;
      |     warning(['Parameter f32IntegGainQ of ' gcb ' exceeds the fixed-point range.']);
      |   end
      |   f32LowerLimitQ=-2147483648;
      |   f32UpperLimitQ=2147483647;
      |   fwkpf=0.9*pgain*wmax/iscale;
      |   s16PropGainShiftFW=ceil(log2(abs(fwkpf)));
      |   if s16PropGainShiftFW<-31
      |     s16PropGainShiftFW=-31;
      |   end
      |   if s16PropGainShiftFW>31
      |     s16PropGainShiftFW=31;
      |     warning(['Parameter s16PropGainShiftFW of ' gcb ' exceeds the fixed-point range.']);
      |   end
      |   f32PropGainFW=round(fwkpf*2^(-s16PropGainShiftFW)*2^31);
      |   if f32PropGainFW>2^31-1
      |     f32PropGainFW=2^31-1;
      |     warning(['Parameter f32PropGainFW of ' gcb ' exceeds the fixed-point range.']);
      |   end
      |   if f32PropGainFW<-2^31
      |     f32PropGainFW=-2^31;
      |     warning(['Parameter f32PropGainFW of ' gcb ' exceeds the fixed-point range.']);
      |   end
      |   s16IntegGainShiftFW=s16IntegGainShiftQ;
      |   f32IntegGainFW=f32IntegGainQ;
      |   if (Idmax<0)
      |     iratio=abs(Idmax)/iscale;
      |     if (abs(iratio) > 1)
      |       iratio = 0;
      |     end
      |     lowlim=0.3183098861837907*acos(iratio)-0.5;
      |   else
      |     lowlim=0.0;
      |   end
      |   f32LowerLimitFW=round(lowlim*2^31);
      |   if f32LowerLimitFW>2^31-1
      |     f32LowerLimitFW=2^31-1;
      |     warning(['Parameter f32LowerLimitFW of ' gcb ' exceeds the fixed-point range.']);
      |   end
      |   if f32LowerLimitFW<-2^31
      |     f32LowerLimitFW=-2^31;
      |     warning(['Parameter f32LowerLimitFW of ' gcb ' exceeds the fixed-point range.']);
      |   end
      |   f32UpperLimitFW=0;
      |   u16NSamplesW=round(log2(1.0/abs(lambdaW)));
      |   if u16NSamplesW>31
      |     u16NSamplesW=31;
      |   end
      |   if u16NSamplesW<0
      |     u16NSamplesW=0;
      |   end
      |   u16NSamplesFW=round(log2(1.0/abs(lambdaFW)));
      |   if u16NSamplesFW>31
      |     u16NSamplesFW=31;
      |   end
      |   if u16NSamplesFW<0
      |     u16NSamplesFW=0;
      |   end
      |   rampsc=polepairs*abs(ramprpm)*0.1047197551196598/wmax;
      |   f32RampUp=round(rampsc*2^31);
      |   if f32RampUp>2^31-1
      |     f32RampUp=2^31-1;
      |     warning(['Parameter f32RampUp of ' gcb ' exceeds the fixed-point range.']);
      |   end
      |   if f32RampUp<-2^31
      |     f32RampUp=-2^31;
      |     warning(['Parameter f32RampUp of ' gcb ' exceeds the fixed-point range.']);
      |   end
      |   f32RampDown=round(rampsc*2^31);
      |   if f32RampDown>2^31-1
      |     f32RampDown=2^31-1;
      |     warning(['Parameter f32RampDown of ' gcb ' exceeds the fixed-point range.']);
      |   end
      |   if f32RampDown<-2^31
      |     f32RampDown=-2^31;
      |     warning(['Parameter f32RampDown of ' gcb ' exceeds the fixed-point range.']);
      |   end
      |   if isnan(u16NSamplesW)
      |     if ~strcmp(u16NSamplesW_bkup,'0')
      |       set_param(gcb,'u16NSamplesW','0');
      |     end
      |   else
      |     tmps=num2str(u16NSamplesW);
      |     if ~strcmp(u16NSamplesW_bkup,tmps)
      |       set_param(gcb,'u16NSamplesW',tmps);
      |     end
      |   end
      |   if isnan(u16NSamplesFW)
      |     if ~strcmp(u16NSamplesFW_bkup,'0')
      |       set_param(gcb,'u16NSamplesFW','0');
      |     end
      |   else
      |     tmps=num2str(u16NSamplesFW);
      |     if ~strcmp(u16NSamplesFW_bkup,tmps)
      |       set_param(gcb,'u16NSamplesFW',tmps);
      |     end
      |   end
      |   if isnan(f32PropGainQ)
      |     if ~strcmp(f32PropGainQ_bkup,'0')
      |       set_param(gcb,'f32PropGainQ','0');
      |     end
      |   else
      |     tmps=num2str(f32PropGainQ);
      |     if ~strcmp(f32PropGainQ_bkup,tmps)
      |       set_param(gcb,'f32PropGainQ',tmps);
      |     end
      |   end
      |   if isnan(f32IntegGainQ)
      |     if ~strcmp(f32IntegGainQ_bkup,'0')
      |       set_param(gcb,'f32IntegGainQ','0');
      |     end
      |   else
      |     tmps=num2str(f32IntegGainQ);
      |     if ~strcmp(f32IntegGainQ_bkup,tmps)
      |       set_param(gcb,'f32IntegGainQ',tmps);
      |     end
      |   end
      |   if isnan(s16PropGainShiftQ)
      |     if ~strcmp(s16PropGainShiftQ_bkup,'0')
      |       set_param(gcb,'s16PropGainShiftQ','0');
      |     end
      |   else
      |     tmps=num2str(s16PropGainShiftQ);
      |     if ~strcmp(s16PropGainShiftQ_bkup,tmps)
      |       set_param(gcb,'s16PropGainShiftQ',tmps);
      |     end
      |   end
      |   if isnan(s16IntegGainShiftQ)
      |     if ~strcmp(s16IntegGainShiftQ_bkup,'0')
      |       set_param(gcb,'s16IntegGainShiftQ','0');
      |     end
      |   else
      |     tmps=num2str(s16IntegGainShiftQ);
      |     if ~strcmp(s16IntegGainShiftQ_bkup,tmps)
      |       set_param(gcb,'s16IntegGainShiftQ',tmps);
      |     end
      |   end
      |   if isnan(f32LowerLimitQ)
      |     if ~strcmp(f32LowerLimitQ_bkup,'0')
      |       set_param(gcb,'f32LowerLimitQ','0');
      |     end
      |   else
      |     tmps=num2str(f32LowerLimitQ);
      |     if ~strcmp(f32LowerLimitQ_bkup,tmps)
      |       set_param(gcb,'f32LowerLimitQ',tmps);
      |     end
      |   end
      |   if isnan(f32UpperLimitQ)
      |     if ~strcmp(f32UpperLimitQ_bkup,'0')
      |       set_param(gcb,'f32UpperLimitQ','0');
      |     end
      |   else
      |     tmps=num2str(f32UpperLimitQ);
      |     if ~strcmp(f32UpperLimitQ_bkup,tmps)
      |       set_param(gcb,'f32UpperLimitQ',tmps);
      |     end
      |   end
      |   if isnan(f32PropGainFW)
      |     if ~strcmp(f32PropGainFW_bkup,'0')
      |       set_param(gcb,'f32PropGainFW','0');
      |     end
      |   else
      |     tmps=num2str(f32PropGainFW);
      |     if ~strcmp(f32PropGainFW_bkup,tmps)
      |       set_param(gcb,'f32PropGainFW',tmps);
      |     end
      |   end
      |   if isnan(f32IntegGainFW)
      |     if ~strcmp(f32IntegGainFW_bkup,'0')
      |       set_param(gcb,'f32IntegGainFW','0');
      |     end
      |   else
      |     tmps=num2str(f32IntegGainFW);
      |     if ~strcmp(f32IntegGainFW_bkup,tmps)
      |       set_param(gcb,'f32IntegGainFW',tmps);
      |     end
      |   end
      |   if isnan(s16PropGainShiftFW)
      |     if ~strcmp(s16PropGainShiftFW_bkup,'0')
      |       set_param(gcb,'s16PropGainShiftFW','0');
      |     end
      |   else
      |     tmps=num2str(s16PropGainShiftFW);
      |     if ~strcmp(s16PropGainShiftFW_bkup,tmps)
      |       set_param(gcb,'s16PropGainShiftFW',tmps);
      |     end
      |   end
      |   if isnan(s16IntegGainShiftFW)
      |     if ~strcmp(s16IntegGainShiftFW_bkup,'0')
      |       set_param(gcb,'s16IntegGainShiftFW','0');
      |     end
      |   else
      |     tmps=num2str(s16IntegGainShiftFW);
      |     if ~strcmp(s16IntegGainShiftFW_bkup,tmps)
      |       set_param(gcb,'s16IntegGainShiftFW',tmps);
      |     end
      |   end
      |   if isnan(f32LowerLimitFW)
      |     if ~strcmp(f32LowerLimitFW_bkup,'0')
      |       set_param(gcb,'f32LowerLimitFW','0');
      |     end
      |   else
      |     tmps=num2str(f32LowerLimitFW);
      |     if ~strcmp(f32LowerLimitFW_bkup,tmps)
      |       set_param(gcb,'f32LowerLimitFW',tmps);
      |     end
      |   end
      |   if isnan(f32UpperLimitFW)
      |     if ~strcmp(f32UpperLimitFW_bkup,'0')
      |       set_param(gcb,'f32UpperLimitFW','0');
      |     end
      |   else
      |     tmps=num2str(f32UpperLimitFW);
      |     if ~strcmp(f32UpperLimitFW_bkup,tmps)
      |       set_param(gcb,'f32UpperLimitFW',tmps);
      |     end
      |   end
      |   if isnan(f32RampUp)
      |     if ~strcmp(f32RampUp_bkup,'0')
      |       set_param(gcb,'f32RampUp','0');
      |     end
      |   else
      |     tmps=num2str(f32RampUp);
      |     if ~strcmp(f32RampUp_bkup,tmps)
      |       set_param(gcb,'f32RampUp',tmps);
      |     end
      |   end
      |   if isnan(f32RampDown)
      |     if ~strcmp(f32RampDown_bkup,'0')
      |       set_param(gcb,'f32RampDown','0');
      |     end
      |   else
      |     tmps=num2str(f32RampDown);
      |     if ~strcmp(f32RampDown_bkup,tmps)
      |       set_param(gcb,'f32RampDown',tmps);
      |     end
      |   end
      | end
      mask Callback polepairs:
      | autoCalcEn=get_param(gcb,'autoCalcEn');
      | if strcmp(autoCalcEn,'on')
      |   SampleTime=Simulink.data.evalinGlobal(bdroot,get_param(gcb,'SampleTime'));
      |   if (SampleTime==-1)
      |     SampleTime=str2double(get_param(gcb,'SampleTime_1'));
      |   end
      |   u16NSamplesW_bkup=get_param(gcb,'u16NSamplesW');
      |   u16NSamplesFW_bkup=get_param(gcb,'u16NSamplesFW');
      |   f32PropGainQ_bkup=get_param(gcb,'f32PropGainQ');
      |   f32IntegGainQ_bkup=get_param(gcb,'f32IntegGainQ');
      |   s16PropGainShiftQ_bkup=get_param(gcb,'s16PropGainShiftQ');
      |   s16IntegGainShiftQ_bkup=get_param(gcb,'s16IntegGainShiftQ');
      |   f32LowerLimitQ_bkup=get_param(gcb,'f32LowerLimitQ');
      |   f32UpperLimitQ_bkup=get_param(gcb,'f32UpperLimitQ');
      |   f32PropGainFW_bkup=get_param(gcb,'f32PropGainFW');
      |   f32IntegGainFW_bkup=get_param(gcb,'f32IntegGainFW');
      |   s16PropGainShiftFW_bkup=get_param(gcb,'s16PropGainShiftFW');
      |   s16IntegGainShiftFW_bkup=get_param(gcb,'s16IntegGainShiftFW');
      |   f32LowerLimitFW_bkup=get_param(gcb,'f32LowerLimitFW');
      |   f32UpperLimitFW_bkup=get_param(gcb,'f32UpperLimitFW');
      |   f32RampUp_bkup=get_param(gcb,'f32RampUp');
      |   f32RampDown_bkup=get_param(gcb,'f32RampDown');
      |   wf0=Simulink.data.evalinGlobal(bdroot,get_param(gcb,'wf0'));
      |   wksi=Simulink.data.evalinGlobal(bdroot,get_param(gcb,'wksi'));
      |   J=Simulink.data.evalinGlobal(bdroot,get_param(gcb,'J'));
      |   Kt=Simulink.data.evalinGlobal(bdroot,get_param(gcb,'Kt'));
      |   lambdaW=Simulink.data.evalinGlobal(bdroot,get_param(gcb,'lambdaW'));
      |   lambdaFW=Simulink.data.evalinGlobal(bdroot,get_param(gcb,'lambdaFW'));
      |   Idmax=Simulink.data.evalinGlobal(bdroot,get_param(gcb,'Idmax'));
      |   ramprpm=Simulink.data.evalinGlobal(bdroot,get_param(gcb,'ramprpm'));
      |   mechspeed=Simulink.data.evalinGlobal(bdroot,get_param(gcb,'mechspeed'));
      |   polepairs=Simulink.data.evalinGlobal(bdroot,get_param(gcb,'polepairs'));
      |   uscale=Simulink.data.evalinGlobal(bdroot,get_param(gcb,'uscale'));
      |   iscale=Simulink.data.evalinGlobal(bdroot,get_param(gcb,'iscale'));
      |   if (wf0<=0)
      |     warning('Natural frequency f0 must be positive.');
      |   end
      |   if (wksi<=0)
      |     warning('Current loop attenuation must be positive.');
      |   end
      |   if (wksi>1)
      |     warning('Current loop attenuation must not exceed 1.');
      |   end
      |   if (J<=0)
      |     warning('Moment of inertia J must be positive.');
      |   end
      |   if (Kt<=0)
      |     warning('Torque constant Kt must be positive.');
      |   end
      |   if (lambdaW<0)
      |     warning('MA filter smoothing factor must be in the range 0..1.');
      |   end
      |   if (lambdaW>1)
      |     warning('MA filter smoothing factor must be in the range 0..1.');
      |   end
      |   if (lambdaFW<0)
      |     warning('MA filter smoothing factor must be in the range 0..1.');
      |   end
      |   if (lambdaFW>1)
      |     warning('MA filter smoothing factor must be in the range 0..1.');
      |   end
      |   if (mechspeed<=0)
      |     warning('Max. speed must be positive.');
      |   end
      |   if (polepairs<1)
      |     warning('Number of pole pairs must be a natural number (1, 2, 3, ...).');
      |   end
      |   if (round(polepairs)~=polepairs)
      |     warning('Number of pole pairs must be a natural number (1, 2, 3, ...).');
      |   end
      |   if (uscale<=0)
      |     warning('U_max must be positive.');
      |   end
      |   if (iscale<=0)
      |     warning('I_max must be positive.');
      |   end
      |   w0=6.283185307179586*wf0;
      |   pgain=2.0*wksi*w0*J/Kt;
      |   igain=w0*w0*J/Kt;
      |   wmax=polepairs*mechspeed*0.1047197551196598;
      |   kpf=pgain*wmax/iscale;
      |   s16PropGainShiftQ=ceil(log2(abs(kpf)));
      |   if s16PropGainShiftQ<-31
      |     s16PropGainShiftQ=-31;
      |   end
      |   if s16PropGainShiftQ>31
      |     s16PropGainShiftQ=31;
      |     warning(['Parameter s16PropGainShiftQ of ' gcb ' exceeds the fixed-point range.']);
      |   end
      |   f32PropGainQ=round(kpf*2^(-s16PropGainShiftQ)*2^31);
      |   if f32PropGainQ>2^31-1
      |     f32PropGainQ=2^31-1;
      |     warning(['Parameter f32PropGainQ of ' gcb ' exceeds the fixed-point range.']);
      |   end
      |   if f32PropGainQ<-2^31
      |     f32PropGainQ=-2^31;
      |     warning(['Parameter f32PropGainQ of ' gcb ' exceeds the fixed-point range.']);
      |   end
      |   kif=igain*SampleTime*0.5*wmax/iscale;
      |   s16IntegGainShiftQ=ceil(log2(abs(kif)));
      |   if s16IntegGainShiftQ<-31
      |     s16IntegGainShiftQ=-31;
      |   end
      |   if s16IntegGainShiftQ>31
      |     s16IntegGainShiftQ=31;
      |     warning(['Parameter s16IntegGainShiftQ of ' gcb ' exceeds the fixed-point range.']);
      |   end
      |   f32IntegGainQ=round(kif*2^(-s16IntegGainShiftQ)*2^31);
      |   if f32IntegGainQ>2^31-1
      |     f32IntegGainQ=2^31-1;
      |     warning(['Parameter f32IntegGainQ of ' gcb ' exceeds the fixed-point range.']);
      |   end
      |   if f32IntegGainQ<-2^31
      |     f32IntegGainQ=-2^31;
      |     warning(['Parameter f32IntegGainQ of ' gcb ' exceeds the fixed-point range.']);
      |   end
      |   f32LowerLimitQ=-2147483648;
      |   f32UpperLimitQ=2147483647;
      |   fwkpf=0.9*pgain*wmax/iscale;
      |   s16PropGainShiftFW=ceil(log2(abs(fwkpf)));
      |   if s16PropGainShiftFW<-31
      |     s16PropGainShiftFW=-31;
      |   end
      |   if s16PropGainShiftFW>31
      |     s16PropGainShiftFW=31;
      |     warning(['Parameter s16PropGainShiftFW of ' gcb ' exceeds the fixed-point range.']);
      |   end
      |   f32PropGainFW=round(fwkpf*2^(-s16PropGainShiftFW)*2^31);
      |   if f32PropGainFW>2^31-1
      |     f32PropGainFW=2^31-1;
      |     warning(['Parameter f32PropGainFW of ' gcb ' exceeds the fixed-point range.']);
      |   end
      |   if f32PropGainFW<-2^31
      |     f32PropGainFW=-2^31;
      |     warning(['Parameter f32PropGainFW of ' gcb ' exceeds the fixed-point range.']);
      |   end
      |   s16IntegGainShiftFW=s16IntegGainShiftQ;
      |   f32IntegGainFW=f32IntegGainQ;
      |   if (Idmax<0)
      |     iratio=abs(Idmax)/iscale;
      |     if (abs(iratio) > 1)
      |       iratio = 0;
      |     end
      |     lowlim=0.3183098861837907*acos(iratio)-0.5;
      |   else
      |     lowlim=0.0;
      |   end
      |   f32LowerLimitFW=round(lowlim*2^31);
      |   if f32LowerLimitFW>2^31-1
      |     f32LowerLimitFW=2^31-1;
      |     warning(['Parameter f32LowerLimitFW of ' gcb ' exceeds the fixed-point range.']);
      |   end
      |   if f32LowerLimitFW<-2^31
      |     f32LowerLimitFW=-2^31;
      |     warning(['Parameter f32LowerLimitFW of ' gcb ' exceeds the fixed-point range.']);
      |   end
      |   f32UpperLimitFW=0;
      |   u16NSamplesW=round(log2(1.0/abs(lambdaW)));
      |   if u16NSamplesW>31
      |     u16NSamplesW=31;
      |   end
      |   if u16NSamplesW<0
      |     u16NSamplesW=0;
      |   end
      |   u16NSamplesFW=round(log2(1.0/abs(lambdaFW)));
      |   if u16NSamplesFW>31
      |     u16NSamplesFW=31;
      |   end
      |   if u16NSamplesFW<0
      |     u16NSamplesFW=0;
      |   end
      |   rampsc=polepairs*abs(ramprpm)*0.1047197551196598/wmax;
      |   f32RampUp=round(rampsc*2^31);
      |   if f32RampUp>2^31-1
      |     f32RampUp=2^31-1;
      |     warning(['Parameter f32RampUp of ' gcb ' exceeds the fixed-point range.']);
      |   end
      |   if f32RampUp<-2^31
      |     f32RampUp=-2^31;
      |     warning(['Parameter f32RampUp of ' gcb ' exceeds the fixed-point range.']);
      |   end
      |   f32RampDown=round(rampsc*2^31);
      |   if f32RampDown>2^31-1
      |     f32RampDown=2^31-1;
      |     warning(['Parameter f32RampDown of ' gcb ' exceeds the fixed-point range.']);
      |   end
      |   if f32RampDown<-2^31
      |     f32RampDown=-2^31;
      |     warning(['Parameter f32RampDown of ' gcb ' exceeds the fixed-point range.']);
      |   end
      |   if isnan(u16NSamplesW)
      |     if ~strcmp(u16NSamplesW_bkup,'0')
      |       set_param(gcb,'u16NSamplesW','0');
      |     end
      |   else
      |     tmps=num2str(u16NSamplesW);
      |     if ~strcmp(u16NSamplesW_bkup,tmps)
      |       set_param(gcb,'u16NSamplesW',tmps);
      |     end
      |   end
      |   if isnan(u16NSamplesFW)
      |     if ~strcmp(u16NSamplesFW_bkup,'0')
      |       set_param(gcb,'u16NSamplesFW','0');
      |     end
      |   else
      |     tmps=num2str(u16NSamplesFW);
      |     if ~strcmp(u16NSamplesFW_bkup,tmps)
      |       set_param(gcb,'u16NSamplesFW',tmps);
      |     end
      |   end
      |   if isnan(f32PropGainQ)
      |     if ~strcmp(f32PropGainQ_bkup,'0')
      |       set_param(gcb,'f32PropGainQ','0');
      |     end
      |   else
      |     tmps=num2str(f32PropGainQ);
      |     if ~strcmp(f32PropGainQ_bkup,tmps)
      |       set_param(gcb,'f32PropGainQ',tmps);
      |     end
      |   end
      |   if isnan(f32IntegGainQ)
      |     if ~strcmp(f32IntegGainQ_bkup,'0')
      |       set_param(gcb,'f32IntegGainQ','0');
      |     end
      |   else
      |     tmps=num2str(f32IntegGainQ);
      |     if ~strcmp(f32IntegGainQ_bkup,tmps)
      |       set_param(gcb,'f32IntegGainQ',tmps);
      |     end
      |   end
      |   if isnan(s16PropGainShiftQ)
      |     if ~strcmp(s16PropGainShiftQ_bkup,'0')
      |       set_param(gcb,'s16PropGainShiftQ','0');
      |     end
      |   else
      |     tmps=num2str(s16PropGainShiftQ);
      |     if ~strcmp(s16PropGainShiftQ_bkup,tmps)
      |       set_param(gcb,'s16PropGainShiftQ',tmps);
      |     end
      |   end
      |   if isnan(s16IntegGainShiftQ)
      |     if ~strcmp(s16IntegGainShiftQ_bkup,'0')
      |       set_param(gcb,'s16IntegGainShiftQ','0');
      |     end
      |   else
      |     tmps=num2str(s16IntegGainShiftQ);
      |     if ~strcmp(s16IntegGainShiftQ_bkup,tmps)
      |       set_param(gcb,'s16IntegGainShiftQ',tmps);
      |     end
      |   end
      |   if isnan(f32LowerLimitQ)
      |     if ~strcmp(f32LowerLimitQ_bkup,'0')
      |       set_param(gcb,'f32LowerLimitQ','0');
      |     end
      |   else
      |     tmps=num2str(f32LowerLimitQ);
      |     if ~strcmp(f32LowerLimitQ_bkup,tmps)
      |       set_param(gcb,'f32LowerLimitQ',tmps);
      |     end
      |   end
      |   if isnan(f32UpperLimitQ)
      |     if ~strcmp(f32UpperLimitQ_bkup,'0')
      |       set_param(gcb,'f32UpperLimitQ','0');
      |     end
      |   else
      |     tmps=num2str(f32UpperLimitQ);
      |     if ~strcmp(f32UpperLimitQ_bkup,tmps)
      |       set_param(gcb,'f32UpperLimitQ',tmps);
      |     end
      |   end
      |   if isnan(f32PropGainFW)
      |     if ~strcmp(f32PropGainFW_bkup,'0')
      |       set_param(gcb,'f32PropGainFW','0');
      |     end
      |   else
      |     tmps=num2str(f32PropGainFW);
      |     if ~strcmp(f32PropGainFW_bkup,tmps)
      |       set_param(gcb,'f32PropGainFW',tmps);
      |     end
      |   end
      |   if isnan(f32IntegGainFW)
      |     if ~strcmp(f32IntegGainFW_bkup,'0')
      |       set_param(gcb,'f32IntegGainFW','0');
      |     end
      |   else
      |     tmps=num2str(f32IntegGainFW);
      |     if ~strcmp(f32IntegGainFW_bkup,tmps)
      |       set_param(gcb,'f32IntegGainFW',tmps);
      |     end
      |   end
      |   if isnan(s16PropGainShiftFW)
      |     if ~strcmp(s16PropGainShiftFW_bkup,'0')
      |       set_param(gcb,'s16PropGainShiftFW','0');
      |     end
      |   else
      |     tmps=num2str(s16PropGainShiftFW);
      |     if ~strcmp(s16PropGainShiftFW_bkup,tmps)
      |       set_param(gcb,'s16PropGainShiftFW',tmps);
      |     end
      |   end
      |   if isnan(s16IntegGainShiftFW)
      |     if ~strcmp(s16IntegGainShiftFW_bkup,'0')
      |       set_param(gcb,'s16IntegGainShiftFW','0');
      |     end
      |   else
      |     tmps=num2str(s16IntegGainShiftFW);
      |     if ~strcmp(s16IntegGainShiftFW_bkup,tmps)
      |       set_param(gcb,'s16IntegGainShiftFW',tmps);
      |     end
      |   end
      |   if isnan(f32LowerLimitFW)
      |     if ~strcmp(f32LowerLimitFW_bkup,'0')
      |       set_param(gcb,'f32LowerLimitFW','0');
      |     end
      |   else
      |     tmps=num2str(f32LowerLimitFW);
      |     if ~strcmp(f32LowerLimitFW_bkup,tmps)
      |       set_param(gcb,'f32LowerLimitFW',tmps);
      |     end
      |   end
      |   if isnan(f32UpperLimitFW)
      |     if ~strcmp(f32UpperLimitFW_bkup,'0')
      |       set_param(gcb,'f32UpperLimitFW','0');
      |     end
      |   else
      |     tmps=num2str(f32UpperLimitFW);
      |     if ~strcmp(f32UpperLimitFW_bkup,tmps)
      |       set_param(gcb,'f32UpperLimitFW',tmps);
      |     end
      |   end
      |   if isnan(f32RampUp)
      |     if ~strcmp(f32RampUp_bkup,'0')
      |       set_param(gcb,'f32RampUp','0');
      |     end
      |   else
      |     tmps=num2str(f32RampUp);
      |     if ~strcmp(f32RampUp_bkup,tmps)
      |       set_param(gcb,'f32RampUp',tmps);
      |     end
      |   end
      |   if isnan(f32RampDown)
      |     if ~strcmp(f32RampDown_bkup,'0')
      |       set_param(gcb,'f32RampDown','0');
      |     end
      |   else
      |     tmps=num2str(f32RampDown);
      |     if ~strcmp(f32RampDown_bkup,tmps)
      |       set_param(gcb,'f32RampDown',tmps);
      |     end
      |   end
      | end
      mask Callback uscale:
      | autoCalcEn=get_param(gcb,'autoCalcEn');
      | if strcmp(autoCalcEn,'on')
      |   SampleTime=Simulink.data.evalinGlobal(bdroot,get_param(gcb,'SampleTime'));
      |   if (SampleTime==-1)
      |     SampleTime=str2double(get_param(gcb,'SampleTime_1'));
      |   end
      |   u16NSamplesW_bkup=get_param(gcb,'u16NSamplesW');
      |   u16NSamplesFW_bkup=get_param(gcb,'u16NSamplesFW');
      |   f32PropGainQ_bkup=get_param(gcb,'f32PropGainQ');
      |   f32IntegGainQ_bkup=get_param(gcb,'f32IntegGainQ');
      |   s16PropGainShiftQ_bkup=get_param(gcb,'s16PropGainShiftQ');
      |   s16IntegGainShiftQ_bkup=get_param(gcb,'s16IntegGainShiftQ');
      |   f32LowerLimitQ_bkup=get_param(gcb,'f32LowerLimitQ');
      |   f32UpperLimitQ_bkup=get_param(gcb,'f32UpperLimitQ');
      |   f32PropGainFW_bkup=get_param(gcb,'f32PropGainFW');
      |   f32IntegGainFW_bkup=get_param(gcb,'f32IntegGainFW');
      |   s16PropGainShiftFW_bkup=get_param(gcb,'s16PropGainShiftFW');
      |   s16IntegGainShiftFW_bkup=get_param(gcb,'s16IntegGainShiftFW');
      |   f32LowerLimitFW_bkup=get_param(gcb,'f32LowerLimitFW');
      |   f32UpperLimitFW_bkup=get_param(gcb,'f32UpperLimitFW');
      |   f32RampUp_bkup=get_param(gcb,'f32RampUp');
      |   f32RampDown_bkup=get_param(gcb,'f32RampDown');
      |   wf0=Simulink.data.evalinGlobal(bdroot,get_param(gcb,'wf0'));
      |   wksi=Simulink.data.evalinGlobal(bdroot,get_param(gcb,'wksi'));
      |   J=Simulink.data.evalinGlobal(bdroot,get_param(gcb,'J'));
      |   Kt=Simulink.data.evalinGlobal(bdroot,get_param(gcb,'Kt'));
      |   lambdaW=Simulink.data.evalinGlobal(bdroot,get_param(gcb,'lambdaW'));
      |   lambdaFW=Simulink.data.evalinGlobal(bdroot,get_param(gcb,'lambdaFW'));
      |   Idmax=Simulink.data.evalinGlobal(bdroot,get_param(gcb,'Idmax'));
      |   ramprpm=Simulink.data.evalinGlobal(bdroot,get_param(gcb,'ramprpm'));
      |   mechspeed=Simulink.data.evalinGlobal(bdroot,get_param(gcb,'mechspeed'));
      |   polepairs=Simulink.data.evalinGlobal(bdroot,get_param(gcb,'polepairs'));
      |   uscale=Simulink.data.evalinGlobal(bdroot,get_param(gcb,'uscale'));
      |   iscale=Simulink.data.evalinGlobal(bdroot,get_param(gcb,'iscale'));
      |   if (wf0<=0)
      |     warning('Natural frequency f0 must be positive.');
      |   end
      |   if (wksi<=0)
      |     warning('Current loop attenuation must be positive.');
      |   end
      |   if (wksi>1)
      |     warning('Current loop attenuation must not exceed 1.');
      |   end
      |   if (J<=0)
      |     warning('Moment of inertia J must be positive.');
      |   end
      |   if (Kt<=0)
      |     warning('Torque constant Kt must be positive.');
      |   end
      |   if (lambdaW<0)
      |     warning('MA filter smoothing factor must be in the range 0..1.');
      |   end
      |   if (lambdaW>1)
      |     warning('MA filter smoothing factor must be in the range 0..1.');
      |   end
      |   if (lambdaFW<0)
      |     warning('MA filter smoothing factor must be in the range 0..1.');
      |   end
      |   if (lambdaFW>1)
      |     warning('MA filter smoothing factor must be in the range 0..1.');
      |   end
      |   if (mechspeed<=0)
      |     warning('Max. speed must be positive.');
      |   end
      |   if (polepairs<1)
      |     warning('Number of pole pairs must be a natural number (1, 2, 3, ...).');
      |   end
      |   if (round(polepairs)~=polepairs)
      |     warning('Number of pole pairs must be a natural number (1, 2, 3, ...).');
      |   end
      |   if (uscale<=0)
      |     warning('U_max must be positive.');
      |   end
      |   if (iscale<=0)
      |     warning('I_max must be positive.');
      |   end
      |   w0=6.283185307179586*wf0;
      |   pgain=2.0*wksi*w0*J/Kt;
      |   igain=w0*w0*J/Kt;
      |   wmax=polepairs*mechspeed*0.1047197551196598;
      |   kpf=pgain*wmax/iscale;
      |   s16PropGainShiftQ=ceil(log2(abs(kpf)));
      |   if s16PropGainShiftQ<-31
      |     s16PropGainShiftQ=-31;
      |   end
      |   if s16PropGainShiftQ>31
      |     s16PropGainShiftQ=31;
      |     warning(['Parameter s16PropGainShiftQ of ' gcb ' exceeds the fixed-point range.']);
      |   end
      |   f32PropGainQ=round(kpf*2^(-s16PropGainShiftQ)*2^31);
      |   if f32PropGainQ>2^31-1
      |     f32PropGainQ=2^31-1;
      |     warning(['Parameter f32PropGainQ of ' gcb ' exceeds the fixed-point range.']);
      |   end
      |   if f32PropGainQ<-2^31
      |     f32PropGainQ=-2^31;
      |     warning(['Parameter f32PropGainQ of ' gcb ' exceeds the fixed-point range.']);
      |   end
      |   kif=igain*SampleTime*0.5*wmax/iscale;
      |   s16IntegGainShiftQ=ceil(log2(abs(kif)));
      |   if s16IntegGainShiftQ<-31
      |     s16IntegGainShiftQ=-31;
      |   end
      |   if s16IntegGainShiftQ>31
      |     s16IntegGainShiftQ=31;
      |     warning(['Parameter s16IntegGainShiftQ of ' gcb ' exceeds the fixed-point range.']);
      |   end
      |   f32IntegGainQ=round(kif*2^(-s16IntegGainShiftQ)*2^31);
      |   if f32IntegGainQ>2^31-1
      |     f32IntegGainQ=2^31-1;
      |     warning(['Parameter f32IntegGainQ of ' gcb ' exceeds the fixed-point range.']);
      |   end
      |   if f32IntegGainQ<-2^31
      |     f32IntegGainQ=-2^31;
      |     warning(['Parameter f32IntegGainQ of ' gcb ' exceeds the fixed-point range.']);
      |   end
      |   f32LowerLimitQ=-2147483648;
      |   f32UpperLimitQ=2147483647;
      |   fwkpf=0.9*pgain*wmax/iscale;
      |   s16PropGainShiftFW=ceil(log2(abs(fwkpf)));
      |   if s16PropGainShiftFW<-31
      |     s16PropGainShiftFW=-31;
      |   end
      |   if s16PropGainShiftFW>31
      |     s16PropGainShiftFW=31;
      |     warning(['Parameter s16PropGainShiftFW of ' gcb ' exceeds the fixed-point range.']);
      |   end
      |   f32PropGainFW=round(fwkpf*2^(-s16PropGainShiftFW)*2^31);
      |   if f32PropGainFW>2^31-1
      |     f32PropGainFW=2^31-1;
      |     warning(['Parameter f32PropGainFW of ' gcb ' exceeds the fixed-point range.']);
      |   end
      |   if f32PropGainFW<-2^31
      |     f32PropGainFW=-2^31;
      |     warning(['Parameter f32PropGainFW of ' gcb ' exceeds the fixed-point range.']);
      |   end
      |   s16IntegGainShiftFW=s16IntegGainShiftQ;
      |   f32IntegGainFW=f32IntegGainQ;
      |   if (Idmax<0)
      |     iratio=abs(Idmax)/iscale;
      |     if (abs(iratio) > 1)
      |       iratio = 0;
      |     end
      |     lowlim=0.3183098861837907*acos(iratio)-0.5;
      |   else
      |     lowlim=0.0;
      |   end
      |   f32LowerLimitFW=round(lowlim*2^31);
      |   if f32LowerLimitFW>2^31-1
      |     f32LowerLimitFW=2^31-1;
      |     warning(['Parameter f32LowerLimitFW of ' gcb ' exceeds the fixed-point range.']);
      |   end
      |   if f32LowerLimitFW<-2^31
      |     f32LowerLimitFW=-2^31;
      |     warning(['Parameter f32LowerLimitFW of ' gcb ' exceeds the fixed-point range.']);
      |   end
      |   f32UpperLimitFW=0;
      |   u16NSamplesW=round(log2(1.0/abs(lambdaW)));
      |   if u16NSamplesW>31
      |     u16NSamplesW=31;
      |   end
      |   if u16NSamplesW<0
      |     u16NSamplesW=0;
      |   end
      |   u16NSamplesFW=round(log2(1.0/abs(lambdaFW)));
      |   if u16NSamplesFW>31
      |     u16NSamplesFW=31;
      |   end
      |   if u16NSamplesFW<0
      |     u16NSamplesFW=0;
      |   end
      |   rampsc=polepairs*abs(ramprpm)*0.1047197551196598/wmax;
      |   f32RampUp=round(rampsc*2^31);
      |   if f32RampUp>2^31-1
      |     f32RampUp=2^31-1;
      |     warning(['Parameter f32RampUp of ' gcb ' exceeds the fixed-point range.']);
      |   end
      |   if f32RampUp<-2^31
      |     f32RampUp=-2^31;
      |     warning(['Parameter f32RampUp of ' gcb ' exceeds the fixed-point range.']);
      |   end
      |   f32RampDown=round(rampsc*2^31);
      |   if f32RampDown>2^31-1
      |     f32RampDown=2^31-1;
      |     warning(['Parameter f32RampDown of ' gcb ' exceeds the fixed-point range.']);
      |   end
      |   if f32RampDown<-2^31
      |     f32RampDown=-2^31;
      |     warning(['Parameter f32RampDown of ' gcb ' exceeds the fixed-point range.']);
      |   end
      |   if isnan(u16NSamplesW)
      |     if ~strcmp(u16NSamplesW_bkup,'0')
      |       set_param(gcb,'u16NSamplesW','0');
      |     end
      |   else
      |     tmps=num2str(u16NSamplesW);
      |     if ~strcmp(u16NSamplesW_bkup,tmps)
      |       set_param(gcb,'u16NSamplesW',tmps);
      |     end
      |   end
      |   if isnan(u16NSamplesFW)
      |     if ~strcmp(u16NSamplesFW_bkup,'0')
      |       set_param(gcb,'u16NSamplesFW','0');
      |     end
      |   else
      |     tmps=num2str(u16NSamplesFW);
      |     if ~strcmp(u16NSamplesFW_bkup,tmps)
      |       set_param(gcb,'u16NSamplesFW',tmps);
      |     end
      |   end
      |   if isnan(f32PropGainQ)
      |     if ~strcmp(f32PropGainQ_bkup,'0')
      |       set_param(gcb,'f32PropGainQ','0');
      |     end
      |   else
      |     tmps=num2str(f32PropGainQ);
      |     if ~strcmp(f32PropGainQ_bkup,tmps)
      |       set_param(gcb,'f32PropGainQ',tmps);
      |     end
      |   end
      |   if isnan(f32IntegGainQ)
      |     if ~strcmp(f32IntegGainQ_bkup,'0')
      |       set_param(gcb,'f32IntegGainQ','0');
      |     end
      |   else
      |     tmps=num2str(f32IntegGainQ);
      |     if ~strcmp(f32IntegGainQ_bkup,tmps)
      |       set_param(gcb,'f32IntegGainQ',tmps);
      |     end
      |   end
      |   if isnan(s16PropGainShiftQ)
      |     if ~strcmp(s16PropGainShiftQ_bkup,'0')
      |       set_param(gcb,'s16PropGainShiftQ','0');
      |     end
      |   else
      |     tmps=num2str(s16PropGainShiftQ);
      |     if ~strcmp(s16PropGainShiftQ_bkup,tmps)
      |       set_param(gcb,'s16PropGainShiftQ',tmps);
      |     end
      |   end
      |   if isnan(s16IntegGainShiftQ)
      |     if ~strcmp(s16IntegGainShiftQ_bkup,'0')
      |       set_param(gcb,'s16IntegGainShiftQ','0');
      |     end
      |   else
      |     tmps=num2str(s16IntegGainShiftQ);
      |     if ~strcmp(s16IntegGainShiftQ_bkup,tmps)
      |       set_param(gcb,'s16IntegGainShiftQ',tmps);
      |     end
      |   end
      |   if isnan(f32LowerLimitQ)
      |     if ~strcmp(f32LowerLimitQ_bkup,'0')
      |       set_param(gcb,'f32LowerLimitQ','0');
      |     end
      |   else
      |     tmps=num2str(f32LowerLimitQ);
      |     if ~strcmp(f32LowerLimitQ_bkup,tmps)
      |       set_param(gcb,'f32LowerLimitQ',tmps);
      |     end
      |   end
      |   if isnan(f32UpperLimitQ)
      |     if ~strcmp(f32UpperLimitQ_bkup,'0')
      |       set_param(gcb,'f32UpperLimitQ','0');
      |     end
      |   else
      |     tmps=num2str(f32UpperLimitQ);
      |     if ~strcmp(f32UpperLimitQ_bkup,tmps)
      |       set_param(gcb,'f32UpperLimitQ',tmps);
      |     end
      |   end
      |   if isnan(f32PropGainFW)
      |     if ~strcmp(f32PropGainFW_bkup,'0')
      |       set_param(gcb,'f32PropGainFW','0');
      |     end
      |   else
      |     tmps=num2str(f32PropGainFW);
      |     if ~strcmp(f32PropGainFW_bkup,tmps)
      |       set_param(gcb,'f32PropGainFW',tmps);
      |     end
      |   end
      |   if isnan(f32IntegGainFW)
      |     if ~strcmp(f32IntegGainFW_bkup,'0')
      |       set_param(gcb,'f32IntegGainFW','0');
      |     end
      |   else
      |     tmps=num2str(f32IntegGainFW);
      |     if ~strcmp(f32IntegGainFW_bkup,tmps)
      |       set_param(gcb,'f32IntegGainFW',tmps);
      |     end
      |   end
      |   if isnan(s16PropGainShiftFW)
      |     if ~strcmp(s16PropGainShiftFW_bkup,'0')
      |       set_param(gcb,'s16PropGainShiftFW','0');
      |     end
      |   else
      |     tmps=num2str(s16PropGainShiftFW);
      |     if ~strcmp(s16PropGainShiftFW_bkup,tmps)
      |       set_param(gcb,'s16PropGainShiftFW',tmps);
      |     end
      |   end
      |   if isnan(s16IntegGainShiftFW)
      |     if ~strcmp(s16IntegGainShiftFW_bkup,'0')
      |       set_param(gcb,'s16IntegGainShiftFW','0');
      |     end
      |   else
      |     tmps=num2str(s16IntegGainShiftFW);
      |     if ~strcmp(s16IntegGainShiftFW_bkup,tmps)
      |       set_param(gcb,'s16IntegGainShiftFW',tmps);
      |     end
      |   end
      |   if isnan(f32LowerLimitFW)
      |     if ~strcmp(f32LowerLimitFW_bkup,'0')
      |       set_param(gcb,'f32LowerLimitFW','0');
      |     end
      |   else
      |     tmps=num2str(f32LowerLimitFW);
      |     if ~strcmp(f32LowerLimitFW_bkup,tmps)
      |       set_param(gcb,'f32LowerLimitFW',tmps);
      |     end
      |   end
      |   if isnan(f32UpperLimitFW)
      |     if ~strcmp(f32UpperLimitFW_bkup,'0')
      |       set_param(gcb,'f32UpperLimitFW','0');
      |     end
      |   else
      |     tmps=num2str(f32UpperLimitFW);
      |     if ~strcmp(f32UpperLimitFW_bkup,tmps)
      |       set_param(gcb,'f32UpperLimitFW',tmps);
      |     end
      |   end
      |   if isnan(f32RampUp)
      |     if ~strcmp(f32RampUp_bkup,'0')
      |       set_param(gcb,'f32RampUp','0');
      |     end
      |   else
      |     tmps=num2str(f32RampUp);
      |     if ~strcmp(f32RampUp_bkup,tmps)
      |       set_param(gcb,'f32RampUp',tmps);
      |     end
      |   end
      |   if isnan(f32RampDown)
      |     if ~strcmp(f32RampDown_bkup,'0')
      |       set_param(gcb,'f32RampDown','0');
      |     end
      |   else
      |     tmps=num2str(f32RampDown);
      |     if ~strcmp(f32RampDown_bkup,tmps)
      |       set_param(gcb,'f32RampDown',tmps);
      |     end
      |   end
      | end
      mask Callback iscale:
      | autoCalcEn=get_param(gcb,'autoCalcEn');
      | if strcmp(autoCalcEn,'on')
      |   SampleTime=Simulink.data.evalinGlobal(bdroot,get_param(gcb,'SampleTime'));
      |   if (SampleTime==-1)
      |     SampleTime=str2double(get_param(gcb,'SampleTime_1'));
      |   end
      |   u16NSamplesW_bkup=get_param(gcb,'u16NSamplesW');
      |   u16NSamplesFW_bkup=get_param(gcb,'u16NSamplesFW');
      |   f32PropGainQ_bkup=get_param(gcb,'f32PropGainQ');
      |   f32IntegGainQ_bkup=get_param(gcb,'f32IntegGainQ');
      |   s16PropGainShiftQ_bkup=get_param(gcb,'s16PropGainShiftQ');
      |   s16IntegGainShiftQ_bkup=get_param(gcb,'s16IntegGainShiftQ');
      |   f32LowerLimitQ_bkup=get_param(gcb,'f32LowerLimitQ');
      |   f32UpperLimitQ_bkup=get_param(gcb,'f32UpperLimitQ');
      |   f32PropGainFW_bkup=get_param(gcb,'f32PropGainFW');
      |   f32IntegGainFW_bkup=get_param(gcb,'f32IntegGainFW');
      |   s16PropGainShiftFW_bkup=get_param(gcb,'s16PropGainShiftFW');
      |   s16IntegGainShiftFW_bkup=get_param(gcb,'s16IntegGainShiftFW');
      |   f32LowerLimitFW_bkup=get_param(gcb,'f32LowerLimitFW');
      |   f32UpperLimitFW_bkup=get_param(gcb,'f32UpperLimitFW');
      |   f32RampUp_bkup=get_param(gcb,'f32RampUp');
      |   f32RampDown_bkup=get_param(gcb,'f32RampDown');
      |   wf0=Simulink.data.evalinGlobal(bdroot,get_param(gcb,'wf0'));
      |   wksi=Simulink.data.evalinGlobal(bdroot,get_param(gcb,'wksi'));
      |   J=Simulink.data.evalinGlobal(bdroot,get_param(gcb,'J'));
      |   Kt=Simulink.data.evalinGlobal(bdroot,get_param(gcb,'Kt'));
      |   lambdaW=Simulink.data.evalinGlobal(bdroot,get_param(gcb,'lambdaW'));
      |   lambdaFW=Simulink.data.evalinGlobal(bdroot,get_param(gcb,'lambdaFW'));
      |   Idmax=Simulink.data.evalinGlobal(bdroot,get_param(gcb,'Idmax'));
      |   ramprpm=Simulink.data.evalinGlobal(bdroot,get_param(gcb,'ramprpm'));
      |   mechspeed=Simulink.data.evalinGlobal(bdroot,get_param(gcb,'mechspeed'));
      |   polepairs=Simulink.data.evalinGlobal(bdroot,get_param(gcb,'polepairs'));
      |   uscale=Simulink.data.evalinGlobal(bdroot,get_param(gcb,'uscale'));
      |   iscale=Simulink.data.evalinGlobal(bdroot,get_param(gcb,'iscale'));
      |   if (wf0<=0)
      |     warning('Natural frequency f0 must be positive.');
      |   end
      |   if (wksi<=0)
      |     warning('Current loop attenuation must be positive.');
      |   end
      |   if (wksi>1)
      |     warning('Current loop attenuation must not exceed 1.');
      |   end
      |   if (J<=0)
      |     warning('Moment of inertia J must be positive.');
      |   end
      |   if (Kt<=0)
      |     warning('Torque constant Kt must be positive.');
      |   end
      |   if (lambdaW<0)
      |     warning('MA filter smoothing factor must be in the range 0..1.');
      |   end
      |   if (lambdaW>1)
      |     warning('MA filter smoothing factor must be in the range 0..1.');
      |   end
      |   if (lambdaFW<0)
      |     warning('MA filter smoothing factor must be in the range 0..1.');
      |   end
      |   if (lambdaFW>1)
      |     warning('MA filter smoothing factor must be in the range 0..1.');
      |   end
      |   if (mechspeed<=0)
      |     warning('Max. speed must be positive.');
      |   end
      |   if (polepairs<1)
      |     warning('Number of pole pairs must be a natural number (1, 2, 3, ...).');
      |   end
      |   if (round(polepairs)~=polepairs)
      |     warning('Number of pole pairs must be a natural number (1, 2, 3, ...).');
      |   end
      |   if (uscale<=0)
      |     warning('U_max must be positive.');
      |   end
      |   if (iscale<=0)
      |     warning('I_max must be positive.');
      |   end
      |   w0=6.283185307179586*wf0;
      |   pgain=2.0*wksi*w0*J/Kt;
      |   igain=w0*w0*J/Kt;
      |   wmax=polepairs*mechspeed*0.1047197551196598;
      |   kpf=pgain*wmax/iscale;
      |   s16PropGainShiftQ=ceil(log2(abs(kpf)));
      |   if s16PropGainShiftQ<-31
      |     s16PropGainShiftQ=-31;
      |   end
      |   if s16PropGainShiftQ>31
      |     s16PropGainShiftQ=31;
      |     warning(['Parameter s16PropGainShiftQ of ' gcb ' exceeds the fixed-point range.']);
      |   end
      |   f32PropGainQ=round(kpf*2^(-s16PropGainShiftQ)*2^31);
      |   if f32PropGainQ>2^31-1
      |     f32PropGainQ=2^31-1;
      |     warning(['Parameter f32PropGainQ of ' gcb ' exceeds the fixed-point range.']);
      |   end
      |   if f32PropGainQ<-2^31
      |     f32PropGainQ=-2^31;
      |     warning(['Parameter f32PropGainQ of ' gcb ' exceeds the fixed-point range.']);
      |   end
      |   kif=igain*SampleTime*0.5*wmax/iscale;
      |   s16IntegGainShiftQ=ceil(log2(abs(kif)));
      |   if s16IntegGainShiftQ<-31
      |     s16IntegGainShiftQ=-31;
      |   end
      |   if s16IntegGainShiftQ>31
      |     s16IntegGainShiftQ=31;
      |     warning(['Parameter s16IntegGainShiftQ of ' gcb ' exceeds the fixed-point range.']);
      |   end
      |   f32IntegGainQ=round(kif*2^(-s16IntegGainShiftQ)*2^31);
      |   if f32IntegGainQ>2^31-1
      |     f32IntegGainQ=2^31-1;
      |     warning(['Parameter f32IntegGainQ of ' gcb ' exceeds the fixed-point range.']);
      |   end
      |   if f32IntegGainQ<-2^31
      |     f32IntegGainQ=-2^31;
      |     warning(['Parameter f32IntegGainQ of ' gcb ' exceeds the fixed-point range.']);
      |   end
      |   f32LowerLimitQ=-2147483648;
      |   f32UpperLimitQ=2147483647;
      |   fwkpf=0.9*pgain*wmax/iscale;
      |   s16PropGainShiftFW=ceil(log2(abs(fwkpf)));
      |   if s16PropGainShiftFW<-31
      |     s16PropGainShiftFW=-31;
      |   end
      |   if s16PropGainShiftFW>31
      |     s16PropGainShiftFW=31;
      |     warning(['Parameter s16PropGainShiftFW of ' gcb ' exceeds the fixed-point range.']);
      |   end
      |   f32PropGainFW=round(fwkpf*2^(-s16PropGainShiftFW)*2^31);
      |   if f32PropGainFW>2^31-1
      |     f32PropGainFW=2^31-1;
      |     warning(['Parameter f32PropGainFW of ' gcb ' exceeds the fixed-point range.']);
      |   end
      |   if f32PropGainFW<-2^31
      |     f32PropGainFW=-2^31;
      |     warning(['Parameter f32PropGainFW of ' gcb ' exceeds the fixed-point range.']);
      |   end
      |   s16IntegGainShiftFW=s16IntegGainShiftQ;
      |   f32IntegGainFW=f32IntegGainQ;
      |   if (Idmax<0)
      |     iratio=abs(Idmax)/iscale;
      |     if (abs(iratio) > 1)
      |       iratio = 0;
      |     end
      |     lowlim=0.3183098861837907*acos(iratio)-0.5;
      |   else
      |     lowlim=0.0;
      |   end
      |   f32LowerLimitFW=round(lowlim*2^31);
      |   if f32LowerLimitFW>2^31-1
      |     f32LowerLimitFW=2^31-1;
      |     warning(['Parameter f32LowerLimitFW of ' gcb ' exceeds the fixed-point range.']);
      |   end
      |   if f32LowerLimitFW<-2^31
      |     f32LowerLimitFW=-2^31;
      |     warning(['Parameter f32LowerLimitFW of ' gcb ' exceeds the fixed-point range.']);
      |   end
      |   f32UpperLimitFW=0;
      |   u16NSamplesW=round(log2(1.0/abs(lambdaW)));
      |   if u16NSamplesW>31
      |     u16NSamplesW=31;
      |   end
      |   if u16NSamplesW<0
      |     u16NSamplesW=0;
      |   end
      |   u16NSamplesFW=round(log2(1.0/abs(lambdaFW)));
      |   if u16NSamplesFW>31
      |     u16NSamplesFW=31;
      |   end
      |   if u16NSamplesFW<0
      |     u16NSamplesFW=0;
      |   end
      |   rampsc=polepairs*abs(ramprpm)*0.1047197551196598/wmax;
